simulink model "ConSys_A1"  (Simulink 8.3)
settings: Solver=ode3  StartTime=0.0  StopTime=Time(end)  FixedStep=Ts  RelTol=1e-3
values from neighbouring files (symbols this model uses):
  d = r*h    (= 1.6)    [StartUp_A1.m]
  d0 = d*h    (= 0.0032)    [StartUp_A1.m]
  h = 0.002    [StartUp_A1.m]
  Ka = diag([ 3  20  20  150  355  520])    [StartUp_A1.m]
  Kd = diag([ 3   5  25  100   15 1050])    [StartUp_A1.m]
  Ki = diag([35 555 810 7410 1850 5815])    [StartUp_A1.m]
  Kp = diag([55 180 350 1960  680 4450])    [StartUp_A1.m]
  r = 800    [StartUp_A1.m]
  TD = ss(Atd,Btd,Ctd,Dtd,Ts)    [StartUp_A1.m]
  Ts = 1/200    (= 0.005)    [StartUp_A1.m]
undefined symbols (not defined in the file or in its folder): DiscIntNeverNeededParam
undefined symbols (not defined in the file): ADAMS_cwd, ADAMS_exec, ADAMS_host, ADAMS_init, ADAMS_inputs, ADAMS_outputs, ADAMS_prefix, ADAMS_static, ADAMS_sysdir
libraries: cstblocks x6
(part 4 of 9)

== matlab function A2/MATLAB Function 1 ==
  data: q input double; V1 output double; dq input double
function V1 = V1(q,dq)
%#codegen
Th1=q(1,1); Th2=q(2,1); Th3=q(3,1); Th4=q(4,1); Th5=q(5,1); Th6=q(6,1);
dTh1=dq(1); dTh2=dq(2); dTh3=dq(3); dTh4=dq(4); dTh5=dq(5); dTh6=dq(6);
%---------------------------
V111=(0)*dTh1*dTh1;
V112=(0.09072*cos(2.0*Th2) + 1.0168*sin(2.0*Th2) + 0.01253*cos(2.0*Th2 + 2.0*Th3) - 0.69402*cos(Th2) - 2.7438*sin(2.0*Th2 + 2.0*Th3) + 0.034055*sin(Th2) + 0.19294*cos(Th2)^2 - 1.0*(1.108*sin(Th2 + Th3) + 4.68*cos(Th2) + 3.302*cos(Th2)*sin(Th3) + 3.302*cos(Th3)*sin(Th2))*(0.08523*cos(Th2 + Th3) - 0.36*sin(Th2) + 0.254*cos(Th2)*cos(Th3) - 0.254*sin(Th2)*sin(Th3) + 0.07) + (cos(Th6)*(sin(Th2 + Th3)*sin(Th5) - 1.0*cos(Th2 + Th3)*cos(Th4)*cos(Th5)) + cos(Th2 + Th3)*sin(Th4)*sin(Th6))*(0.001043*cos(Th6)*(cos(Th2 + Th3)*sin(Th5) + sin(Th2 + Th3)*cos(Th4)*cos(Th5)) - 4.0e-6*cos(Th2 + Th3)*cos(Th5) + 4.0e-6*sin(Th2 + Th3)*cos(Th4)*sin(Th5) - 0.001043*sin(Th2 + Th3)*sin(Th4)*sin(Th6)) + 0.009886*cos(Th2 + Th3)*sin(Th2 + Th3) + (sin(Th6)*(cos(Th2 + Th3)*sin(Th5) + sin(Th2 + Th3)*cos(Th4)*cos(Th5)) + sin(Th2 + Th3)*cos(Th6)*sin(Th4))*(0.00104*sin(Th6)*(sin(Th2 + Th3)*sin(Th5) - 1.0*cos(Th2 + Th3)*cos(Th4)*cos(Th5)) - 0.00104*cos(Th2 + Th3)*cos(Th6)*sin(Th4)) + (sin(Th6)*(sin(Th2 + Th3)*sin(Th5) - 1.0*cos(Th2 + Th3)*cos(Th4)*cos(Th5)) - 1.0*cos(Th2 + Th3)*cos(Th6)*sin(Th4))*(0.00104*sin(Th6)*(cos(Th2 + Th3)*sin(Th5) + sin(Th2 + Th3)*cos(Th4)*cos(Th5)) + 0.00104*sin(Th2 + Th3)*cos(Th6)*sin(Th4)) - 1.0*(sin(Th2 + Th3)*cos(Th5) + cos(Th2 + Th3)*cos(Th4)*sin(Th5))*(4.0e-6*cos(Th6)*(cos(Th2 + Th3)*sin(Th5) + sin(Th2 + Th3)*cos(Th4)*cos(Th5)) - 0.000116*cos(Th2 + Th3)*cos(Th5) + 0.000116*sin(Th2 + Th3)*cos(Th4)*sin(Th5) - 4.0e-6*sin(Th2 + Th3)*sin(Th4)*sin(Th6)) - 1.0*(cos(Th2 + Th3)*cos(Th5) - 1.0*sin(Th2 + Th3)*cos(Th4)*sin(Th5))*(4.0e-6*cos(Th6)*(sin(Th2 + Th3)*sin(Th5) - 1.0*cos(Th2 + Th3)*cos(Th4)*cos(Th5)) - 0.000116*sin(Th2 + Th3)*cos(Th5) - 0.000116*cos(Th2 + Th3)*cos(Th4)*sin(Th5) + 4.0e-6*cos(Th2 + Th3)*sin(Th4)*sin(Th6)) + (0.252*sin(Th2 + Th3) + 0.72*cos(Th2) + 0.00124*cos(Th2 + Th3)*sin(Th4) - 0.00304*sin(Th2 + Th3)*cos(Th5) - 0.00004*sin(Th2 + Th3)*sin(Th5) + 0.508*cos(Th2)*sin(Th3) + 0.508*cos(Th3)*sin(Th2) + 0.00004*cos(Th2 + Th3)*cos(Th4)*cos(Th5) - 0.00304*cos(Th2 + Th3)*cos(Th4)*sin(Th5))*(0.36*sin(Th2) - 0.126*cos(Th2 + Th3) + 0.00152*cos(Th2 + Th3)*cos(Th5) + 0.00002*cos(Th2 + Th3)*sin(Th5) + 0.00062*sin(Th2 + Th3)*sin(Th4) - 0.254*cos(Th2)*cos(Th3) + 0.254*sin(Th2)*sin(Th3) + 0.00002*sin(Th2 + Th3)*cos(Th4)*cos(Th5) - 0.00152*sin(Th2 + Th3)*cos(Th4)*sin(Th5) - 0.07) - 1.0*(0.126*sin(Th2 + Th3) + 0.36*cos(Th2) + 0.05206*sin(Th2 + Th3)*cos(Th5) + 0.254*cos(Th2)*sin(Th3) + 0.254*cos(Th3)*sin(Th2) + 0.05206*cos(Th2 + Th3)*cos(Th4)*sin(Th5) + 0.00023*cos(Th2 + Th3)*sin(Th4)*sin(Th6) + 0.00023*sin(Th2 + Th3)*cos(Th6)*sin(Th5) - 0.00023*cos(Th2 + Th3)*cos(Th4)*cos(Th5)*cos(Th6))*(0.126*cos(Th2 + Th3) - 0.36*sin(Th2) + 0.05206*cos(Th2 + Th3)*cos(Th5) + 0.254*cos(Th2)*cos(Th3) - 0.254*sin(Th2)*sin(Th3) + 0.00023*cos(Th2 + Th3)*cos(Th6)*sin(Th5) - 0.05206*sin(Th2 + Th3)*cos(Th4)*sin(Th5) - 0.00023*sin(Th2 + Th3)*sin(Th4)*sin(Th6) + 0.00023*sin(Th2 + Th3)*cos(Th4)*cos(Th5)*cos(Th6) + 0.07) - 1.0*(0.03204*cos(Th2 + Th3) + 4.9136*sin(Th2 + Th3) - 12.96*cos(Th2))*(0.13649*cos(Th2 + Th3) - 0.00089*sin(Th2 + Th3) + 0.36*sin(Th2) - 0.07) + 1.9612*cos(Th2)*sin(Th2) + (cos(Th6)*(cos(Th2 + Th3)*sin(Th5) + sin(Th2 + Th3)*cos(Th4)*cos(Th5)) - 1.0*sin(Th2 + Th3)*sin(Th4)*sin(Th6))*(0.001043*cos(Th6)*(sin(Th2 + Th3)*sin(Th5) - 1.0*cos(Th2 + Th3)*cos(Th4)*cos(Th5)) - 4.0e-6*sin(Th2 + Th3)*cos(Th5) - 4.0e-6*cos(Th2 + Th3)*cos(Th4)*sin(Th5) + 0.001043*cos(Th2 + Th3)*sin(Th4)*sin(Th6)) - 0.02225*cos(Th2 + Th3)*sin(Th2 + Th3)*cos(Th4)^2 + 0.000978*cos(Th2 + Th3)*sin(Th2 + Th3)*cos(Th5)^2 - 0.04182*cos(Th2 + Th3)*sin(Th2 + Th3)*sin(Th4)^2 + 0.009796*cos(Th2 + Th3)*sin(Th2 + Th3)*sin(Th5)^2 - 0.00008*cos(Th2 + Th3)^2*cos(Th5)*sin(Th4) + 0.00008*sin(Th2 + Th3)^2*cos(Th5)*sin(Th4) - 0.008818*cos(Th2 + Th3)^2*cos(Th4)*cos(Th5)*sin(Th5) + 0.008818*sin(Th2 + Th3)^2*cos(Th4)*cos(Th5)*sin(Th5) - 0.009796*cos(Th2 + Th3)*sin(Th2 + Th3)*cos(Th4)^2*cos(Th5)^2 - 0.000978*cos(Th2 + Th3)*sin(Th2 + Th3)*cos(Th4)^2*sin(Th5)^2 + 0.00016*cos(Th2 + Th3)*sin(Th2 + Th3)*cos(Th4)*sin(Th4)*sin(Th5) - 0.096468)*dTh1*dTh2;
V113=(0.01253*cos(2.0*Th2 + 2.0*Th3) - 2.7438*sin(2.0*Th2 + 2.0*Th3) - 1.0*(0.03204*cos(Th2 + Th3) + 4.9136*sin(Th2 + Th3))*(0.13649*cos(Th2 + Th3) - 0.00089*sin(Th2 + Th3) + 0.36*sin(Th2) - 0.07) + (cos(Th6)*(sin(Th2 + Th3)*sin(Th5) - 1.0*cos(Th2 + Th3)*cos(Th4)*cos(Th5)) + cos(Th2 + Th3)*sin(Th4)*sin(Th6))*(0.001043*cos(Th6)*(cos(Th2 + Th3)*sin(Th5) + sin(Th2 + Th3)*cos(Th4)*cos(Th5)) - 4.0e-6*cos(Th2 + Th3)*cos(Th5) + 4.0e-6*sin(Th2 + Th3)*cos(Th4)*sin(Th5) - 0.001043*sin(Th2 + Th3)*sin(Th4)*sin(Th6)) + (0.252*sin(Th2 + Th3) + 0.00124*cos(Th2 + Th3)*sin(Th4) - 0.00304*sin(Th2 + Th3)*cos(Th5) - 0.00004*sin(Th2 + Th3)*sin(Th5) + 0.508*cos(Th2)*sin(Th3) + 0.508*cos(Th3)*sin(Th2) + 0.00004*cos(Th2 + Th3)*cos(Th4)*cos(Th5) - 0.00304*cos(Th2 + Th3)*cos(Th4)*sin(Th5))*(0.36*sin(Th2) - 0.126*cos(Th2 + Th3) + 0.00152*cos(Th2 + Th3)*cos(Th5) + 0.00002*cos(Th2 + Th3)*sin(Th5) + 0.00062*sin(Th2 + Th3)*sin(Th4) - 0.254*cos(Th2)*cos(Th3) + 0.254*sin(Th2)*sin(Th3) + 0.00002*sin(Th2 + Th3)*cos(Th4)*cos(Th5) - 0.00152*sin(Th2 + Th3)*cos(Th4)*sin(Th5) - 0.07) - 1.0*(0.126*sin(Th2 + Th3) + 0.05206*sin(Th2 + Th3)*cos(Th5) + 0.254*cos(Th2)*sin(Th3) + 0.254*cos(Th3)*sin(Th2) + 0.05206*cos(Th2 + Th3)*cos(Th4)*sin(Th5) + 0.00023*cos(Th2 + Th3)*sin(Th4)*sin(Th6) + 0.00023*sin(Th2 + Th3)*cos(Th6)*sin(Th5) - 0.00023*cos(Th2 + Th3)*cos(Th4)*cos(Th5)*cos(Th6))*(0.126*cos(Th2 + Th3) - 0.36*sin(Th2) + 0.05206*cos(Th2 + Th3)*cos(Th5) + 0.254*cos(Th2)*cos(Th3) - 0.254*sin(Th2)*sin(Th3) + 0.00023*cos(Th2 + Th3)*cos(Th6)*sin(Th5) - 0.05206*sin(Th2 + Th3)*cos(Th4)*sin(Th5) - 0.00023*sin(Th2 + Th3)*sin(Th4)*sin(Th6) + 0.00023*sin(Th2 + Th3)*cos(Th4)*cos(Th5)*cos(Th6) + 0.07) + 0.009886*cos(Th2 + Th3)*sin(Th2 + Th3) + (sin(Th6)*(cos(Th2 + Th3)*sin(Th5) + sin(Th2 + Th3)*cos(Th4)*cos(Th5)) + sin(Th2 + Th3)*cos(Th6)*sin(Th4))*(0.00104*sin(Th6)*(sin(Th2 + Th3)*sin(Th5) - 1.0*cos(Th2 + Th3)*cos(Th4)*cos(Th5)) - 0.00104*cos(Th2 + Th3)*cos(Th6)*sin(Th4)) + (sin(Th6)*(sin(Th2 + Th3)*sin(Th5) - 1.0*cos(Th2 + Th3)*cos(Th4)*cos(Th5)) - 1.0*cos(Th2 + Th3)*cos(Th6)*sin(Th4))*(0.00104*sin(Th6)*(cos(Th2 + Th3)*sin(Th5) + sin(Th2 + Th3)*cos(Th4)*cos(Th5)) + 0.00104*sin(Th2 + Th3)*cos(Th6)*sin(Th4)) - 1.0*(sin(Th2 + Th3)*cos(Th5) + cos(Th2 + Th3)*cos(Th4)*sin(Th5))*(4.0e-6*cos(Th6)*(cos(Th2 + Th3)*sin(Th5) + sin(Th2 + Th3)*cos(Th4)*cos(Th5)) - 0.000116*cos(Th2 + Th3)*cos(Th5) + 0.000116*sin(Th2 + Th3)*cos(Th4)*sin(Th5) - 4.0e-6*sin(Th2 + Th3)*sin(Th4)*sin(Th6)) - 1.0*(cos(Th2 + Th3)*cos(Th5) - 1.0*sin(Th2 + Th3)*cos(Th4)*sin(Th5))*(4.0e-6*cos(Th6)*(sin(Th2 + Th3)*sin(Th5) - 1.0*cos(Th2 + Th3)*cos(Th4)*cos(Th5)) - 0.000116*sin(Th2 + Th3)*cos(Th5) - 0.000116*cos(Th2 + Th3)*cos(Th4)*sin(Th5) + 4.0e-6*cos(Th2 + Th3)*sin(Th4)*sin(Th6)) - 1.0*(1.108*sin(Th2 + Th3) + 3.302*cos(Th2)*sin(Th3) + 3.302*cos(Th3)*sin(Th2))*(0.08523*cos(Th2 + Th3) - 0.36*sin(Th2) + 0.254*cos(Th2)*cos(Th3) - 0.254*sin(Th2)*sin(Th3) + 0.07) + (cos(Th6)*(cos(Th2 + Th3)*sin(Th5) + sin(Th2 + Th3)*cos(Th4)*cos(Th5)) - 1.0*sin(Th2 + Th3)*sin(Th4)*sin(Th6))*(0.001043*cos(Th6)*(sin(Th2 + Th3)*sin(Th5) - 1.0*cos(Th2 + Th3)*cos(Th4)*cos(Th5)) - 4.0e-6*sin(Th2 + Th3)*cos(Th5) - 4.0e-6*cos(Th2 + Th3)*cos(Th4)*sin(Th5) + 0.001043*cos(Th2 + Th3)*sin(Th4)*sin(Th6)) - 0.02225*cos(Th2 + Th3)*sin(Th2 + Th3)*cos(Th4)^2 + 0.000978*cos(Th2 + Th3)*sin(Th2 + Th3)*cos(Th5)^2 - 0.04182*cos(Th2 + Th3)*sin(Th2 + Th3)*sin(Th4)^2 + 0.009796*cos(Th2 + Th3)*sin(Th2 + Th3)*sin(Th5)^2 - 0.00008*cos(Th2 + Th3)^2*cos(Th5)*sin(Th4) + 0.00008*sin(Th2 + Th3)^2*cos(Th5)*sin(Th4) - 0.008818*cos(Th2 + Th3)^2*cos(Th4)*cos(Th5)*sin(Th5) + 0.008818*sin(Th2 + Th3)^2*cos(Th4)*cos(Th5)*sin(Th5) - 0.009796*cos(Th2 + Th3)*sin(Th2 + Th3)*cos(Th4)^2*cos(Th5)^2 - 0.000978*cos(Th2 + Th3)*sin(Th2 + Th3)*cos(Th4)^2*sin(Th5)^2 + 0.00016*cos(Th2 + Th3)*sin(Th2 + Th3)*cos(Th4)*sin(Th4)*sin(Th5))*dTh1*dTh3;
V114=((0.00124*cos(Th4) - 0.00004*cos(Th5)*sin(Th4) + 0.00304*sin(Th4)*sin(Th5))*(0.00062*sin(Th2 + Th3)^2*sin(Th4) - 0.063*sin(2.0*Th2 + 2.0*Th3) - 0.00062*sin(Th4) - 0.07*sin(Th2 + Th3) + 0.36*sin(Th2 + Th3)*sin(Th2) - 0.00002*cos(Th4)*cos(Th5) + 0.00152*cos(Th4)*sin(Th5) + 0.00002*cos(Th2 + Th3)*sin(Th2 + Th3)*sin(Th5) - 0.254*sin(Th2 + Th3)*cos(Th2)*cos(Th3) + 0.254*sin(Th2 + Th3)*sin(Th2)*sin(Th3) + 0.00002*sin(Th2 + Th3)^2*cos(Th4)*cos(Th5) - 0.00152*sin(Th2 + Th3)^2*cos(Th4)*sin(Th5) + 0.00152*cos(Th2 + Th3)*sin(Th2 + Th3)*cos(Th5)) - 1.0*(0.00023*cos(Th4)*sin(Th6) - 0.05206*sin(Th4)*sin(Th5) + 0.00023*cos(Th5)*cos(Th6)*sin(Th4))*(0.07*sin(Th2 + Th3) + 0.063*sin(2.0*Th2 + 2.0*Th3) - 0.36*sin(Th2 + Th3)*sin(Th2) + 0.05206*cos(Th4)*sin(Th5) + 0.00023*sin(Th4)*sin(Th6) + 0.254*sin(Th2 + Th3)*cos(Th2)*cos(Th3) - 0.254*sin(Th2 + Th3)*sin(Th2)*sin(Th3) - 0.00023*cos(Th4)*cos(Th5)*cos(Th6) - 0.05206*sin(Th2 + Th3)^2*cos(Th4)*sin(Th5) - 0.00023*sin(Th2 + Th3)^2*sin(Th4)*sin(Th6) + 0.05206*cos(Th2 + Th3)*sin(Th2 + Th3)*cos(Th5) + 0.00023*sin(Th2 + Th3)^2*cos(Th4)*cos(Th5)*cos(Th6) + 0.00023*cos(Th2 + Th3)*sin(Th2 + Th3)*cos(Th6)*sin(Th5)) + 2.2737e-18*cos(Th2 + Th3)*(3.5184e13*cos(Th2 + Th3)*sin(Th5) + 4.1368e15*cos(Th2 + Th3)*cos(Th4)*sin(Th4) - 3.5184e13*sin(Th2 + Th3)*cos(Th4)*cos(Th5) - 7.0369e13*cos(Th2 + Th3)*cos(Th4)^2*sin(Th5) + 3.8782e15*sin(Th2 + Th3)*cos(Th5)*sin(Th4)*sin(Th5) - 3.8782e15*cos(Th2 + Th3)*cos(Th4)*cos(Th5)^2*sin(Th4)) + 8.4703e-22*cos(Th2 + Th3)*(1.2314e18*cos(Th4)*sin(Th6) + 4.7224e15*sin(Th4)*sin(Th5) + 1.2314e18*cos(Th5)*cos(Th6)*sin(Th4))*(cos(Th2 + Th3)*sin(Th4)*sin(Th6) + sin(Th2 + Th3)*cos(Th6)*sin(Th5) - 1.0*cos(Th2 + Th3)*cos(Th4)*cos(Th5)*cos(Th6)) + 0.00104*cos(Th2 + Th3)*(cos(Th4)*cos(Th6) - 1.0*cos(Th5)*sin(Th4)*sin(Th6))*(cos(Th2 + Th3)*cos(Th6)*sin(Th4) - 1.0*sin(Th2 + Th3)*sin(Th5)*sin(Th6) + cos(Th2 + Th3)*cos(Th4)*cos(Th5)*sin(Th6)) + 0.009186*cos(Th2 + Th3)^2*cos(Th4)*sin(Th4) + cos(Th2 + Th3)*(cos(Th4)*cos(Th6) - 1.0*cos(Th5)*sin(Th4)*sin(Th6))*(0.00104*cos(Th2 + Th3)*cos(Th6)*sin(Th4) - 0.00104*sin(Th2 + Th3)*sin(Th5)*sin(Th6) + 0.00104*cos(Th2 + Th3)*cos(Th4)*cos(Th5)*sin(Th6)) - 1.0*cos(Th2 + Th3)*(cos(Th4)*sin(Th6) + cos(Th5)*cos(Th6)*sin(Th4))*(4.0e-6*sin(Th2 + Th3)*cos(Th5) + 4.0e-6*cos(Th2 + Th3)*cos(Th4)*sin(Th5) - 0.001043*cos(Th2 + Th3)*sin(Th4)*sin(Th6) - 0.001043*sin(Th2 + Th3)*cos(Th6)*sin(Th5) + 0.001043*cos(Th2 + Th3)*cos(Th4)*cos(Th5)*cos(Th6)) - 8.4703e-22*cos(Th2 + Th3)*(sin(Th2 + Th3)*cos(Th5) + cos(Th2 + Th3)*cos(Th4)*sin(Th5))*(4.7224e15*cos(Th4)*sin(Th6) + 1.3695e17*sin(Th4)*sin(Th5) + 4.7224e15*cos(Th5)*cos(Th6)*sin(Th4)) - 1.0*cos(Th2 + Th3)*sin(Th4)*sin(Th5)*(0.000116*sin(Th2 + Th3)*cos(Th5) + 0.000116*cos(Th2 + Th3)*cos(Th4)*sin(Th5) - 4.0e-6*cos(Th2 + Th3)*sin(Th4)*sin(Th6) - 4.0e-6*sin(Th2 + Th3)*cos(Th6)*sin(Th5) + 4.0e-6*cos(Th2 + Th3)*cos(Th4)*cos(Th5)*cos(Th6)))*dTh1*dTh4;
V115=((cos(Th6)*(sin(Th2 + Th3)*sin(Th5) - 1.0*cos(Th2 + Th3)*cos(Th4)*cos(Th5)) + cos(Th2 + Th3)*sin(Th4)*sin(Th6))*(0.001043*cos(Th6)*(sin(Th2 + Th3)*cos(Th5) + cos(Th2 + Th3)*cos(Th4)*sin(Th5)) + 4.0e-6*sin(Th2 + Th3)*sin(Th5) - 4.0e-6*cos(Th2 + Th3)*cos(Th4)*cos(Th5)) - 1.0*(sin(Th2 + Th3)*cos(Th5) + cos(Th2 + Th3)*cos(Th4)*sin(Th5))*(4.0e-6*cos(Th6)*(sin(Th2 + Th3)*cos(Th5) + cos(Th2 + Th3)*cos(Th4)*sin(Th5)) + 0.000116*sin(Th2 + Th3)*sin(Th5) - 0.000116*cos(Th2 + Th3)*cos(Th4)*cos(Th5)) + (sin(Th2 + Th3)*sin(Th5) - 1.0*cos(Th2 + Th3)*cos(Th4)*cos(Th5))*(4.0e-6*cos(Th6)*(sin(Th2 + Th3)*sin(Th5) - 1.0*cos(Th2 + Th3)*cos(Th4)*cos(Th5)) - 0.000116*sin(Th2 + Th3)*cos(Th5) - 0.000116*cos(Th2 + Th3)*cos(Th4)*sin(Th5) + 4.0e-6*cos(Th2 + Th3)*sin(Th4)*sin(Th6)) + (0.00023*cos(Th6)*(sin(Th5)*(sin(Th1)*sin(Th4) - 1.0*sin(Th2 + Th3)*cos(Th1)*cos(Th4)) + cos(Th2 + Th3)*cos(Th1)*cos(Th5)) + 0.05206*cos(Th5)*(sin(Th1)*sin(Th4) - 1.0*sin(Th2 + Th3)*cos(Th1)*cos(Th4)) - 0.05206*cos(Th2 + Th3)*cos(Th1)*sin(Th5))*(0.07*cos(Th1) + 0.05206*sin(Th5)*(sin(Th1)*sin(Th4) - 1.0*sin(Th2 + Th3)*cos(Th1)*cos(Th4)) + 0.126*cos(Th2 + Th3)*cos(Th1) - 0.00023*sin(Th6)*(cos(Th4)*sin(Th1) + sin(Th2 + Th3)*cos(Th1)*sin(Th4)) - 0.36*cos(Th1)*sin(Th2) - 0.00023*cos(Th6)*(cos(Th5)*(sin(Th1)*sin(Th4) - 1.0*sin(Th2 + Th3)*cos(Th1)*cos(Th4)) - 1.0*cos(Th2 + Th3)*cos(Th1)*sin(Th5)) + 0.05206*cos(Th2 + Th3)*cos(Th1)*cos(Th5) + 0.254*cos(Th1)*cos(Th2)*cos(Th3) - 0.254*cos(Th1)*sin(Th2)*sin(Th3)) - 1.0*(0.00304*cos(Th5)*(cos(Th1)*sin(Th4) + sin(Th2 + Th3)*cos(Th4)*sin(Th1)) + 0.00004*sin(Th5)*(cos(Th1)*sin(Th4) + sin(Th2 + Th3)*cos(Th4)*sin(Th1)) - 0.00004*cos(Th2 + Th3)*cos(Th5)*sin(Th1) + 0.00304*cos(Th2 + Th3)*sin(Th1)*sin(Th5))*(0.00002*cos(Th5)*(cos(Th1)*sin(Th4) + sin(Th2 + Th3)*cos(Th4)*sin(Th1)) - 0.126*cos(Th2 + Th3)*sin(Th1) - 0.07*sin(Th1) - 0.00152*sin(Th5)*(cos(Th1)*sin(Th4) + sin(Th2 + Th3)*cos(Th4)*sin(Th1)) - 0.00062*cos(Th1)*cos(Th4) + 0.36*sin(Th1)*sin(Th2) + 0.00152*cos(Th2 + Th3)*cos(Th5)*sin(Th1) + 0.00002*cos(Th2 + Th3)*sin(Th1)*sin(Th5) + 0.00062*sin(Th2 + Th3)*sin(Th1)*sin(Th4) - 0.254*cos(Th2)*cos(Th3)*sin(Th1) + 0.254*sin(Th1)*sin(Th2)*sin(Th3)) + (0.00304*cos(Th5)*(sin(Th1)*sin(Th4) - 1.0*sin(Th2 + Th3)*cos(Th1)*cos(Th4)) + 0.00004*sin(Th5)*(sin(Th1)*sin(Th4) - 1.0*sin(Th2 + Th3)*cos(Th1)*cos(Th4)) + 0.00004*cos(Th2 + Th3)*cos(Th1)*cos(Th5) - 0.00304*cos(Th2 + Th3)*cos(Th1)*sin(Th5))*(0.00152*sin(Th5)*(sin(Th1)*sin(Th4) - 1.0*sin(Th2 + Th3)*cos(Th1)*cos(Th4)) - 0.00002*cos(Th5)*(sin(Th1)*sin(Th4) - 1.0*sin(Th2 + Th3)*cos(Th1)*cos(Th4)) - 0.07*cos(Th1) - 0.126*cos(Th2 + Th3)*cos(Th1) + 0.36*cos(Th1)*sin(Th2) + 0.00062*cos(Th4)*sin(Th1) + 0.00152*cos(Th2 + Th3)*cos(Th1)*cos(Th5) + 0.00002*cos(Th2 + Th3)*cos(Th1)*sin(Th5) + 0.00062*sin(Th2 + Th3)*cos(Th1)*sin(Th4) - 0.254*cos(Th1)*cos(Th2)*cos(Th3) + 0.254*cos(Th1)*sin(Th2)*sin(Th3)) - 1.0*(0.00023*cos(Th6)*(sin(Th5)*(cos(Th1)*sin(Th4) + sin(Th2 + Th3)*cos(Th4)*sin(Th1)) - 1.0*cos(Th2 + Th3)*cos(Th5)*sin(Th1)) + 0.05206*cos(Th5)*(cos(Th1)*sin(Th4) + sin(Th2 + Th3)*cos(Th4)*sin(Th1)) + 0.05206*cos(Th2 + Th3)*sin(Th1)*sin(Th5))*(0.07*sin(Th1) + 0.00023*sin(Th6)*(cos(Th1)*cos(Th4) - 1.0*sin(Th2 + Th3)*sin(Th1)*sin(Th4)) + 0.00023*cos(Th6)*(cos(Th5)*(cos(Th1)*sin(Th4) + sin(Th2 + Th3)*cos(Th4)*sin(Th1)) + cos(Th2 + Th3)*sin(Th1)*sin(Th5)) + 0.126*cos(Th2 + Th3)*sin(Th1) - 0.05206*sin(Th5)*(cos(Th1)*sin(Th4) + sin(Th2 + Th3)*cos(Th4)*sin(Th1)) - 0.36*sin(Th1)*sin(Th2) + 0.05206*cos(Th2 + Th3)*cos(Th5)*sin(Th1) + 0.254*cos(Th2)*cos(Th3)*sin(Th1) - 0.254*sin(Th1)*sin(Th2)*sin(Th3)) + cos(Th6)*(sin(Th2 + Th3)*cos(Th5) + cos(Th2 + Th3)*cos(Th4)*sin(Th5))*(0.001043*cos(Th6)*(sin(Th2 + Th3)*sin(Th5) - 1.0*cos(Th2 + Th3)*cos(Th4)*cos(Th5)) - 4.0e-6*sin(Th2 + Th3)*cos(Th5) - 4.0e-6*cos(Th2 + Th3)*cos(Th4)*sin(Th5) + 0.001043*cos(Th2 + Th3)*sin(Th4)*sin(Th6)) + sin(Th6)*(sin(Th2 + Th3)*cos(Th5) + cos(Th2 + Th3)*cos(Th4)*sin(Th5))*(0.00104*sin(Th6)*(sin(Th2 + Th3)*sin(Th5) - 1.0*cos(Th2 + Th3)*cos(Th4)*cos(Th5)) - 0.00104*cos(Th2 + Th3)*cos(Th6)*sin(Th4)) + 0.008818*sin(Th2 + Th3)^2*cos(Th5)*sin(Th5) + 0.00104*sin(Th6)*(sin(Th2 + Th3)*cos(Th5) + cos(Th2 + Th3)*cos(Th4)*sin(Th5))*(sin(Th6)*(sin(Th2 + Th3)*sin(Th5) - 1.0*cos(Th2 + Th3)*cos(Th4)*cos(Th5)) - 1.0*cos(Th2 + Th3)*cos(Th6)*sin(Th4)) - 0.008818*cos(Th2 + Th3)*sin(Th2 + Th3)*cos(Th4)*cos(Th5)^2 + 0.008818*cos(Th2 + Th3)*sin(Th2 + Th3)*cos(Th4)*sin(Th5)^2 - 0.00008*cos(Th2 + Th3)^2*cos(Th4)*cos(Th5)*sin(Th4) - 0.008818*cos(Th2 + Th3)^2*cos(Th4)^2*cos(Th5)*sin(Th5) + 0.00008*cos(Th2 + Th3)*sin(Th2 + Th3)*sin(Th4)*sin(Th5))*dTh1*dTh5;
V116=(1.0*(0.00023*cos(Th6)*(cos(Th1)*cos(Th4) - 1.0*sin(Th2 + Th3)*sin(Th1)*sin(Th4)) - 0.00023*sin(Th6)*(cos(Th5)*(cos(Th1)*sin(Th4) + sin(Th2 + Th3)*cos(Th4)*sin(Th1)) + cos(Th2 + Th3)*sin(Th1)*sin(Th5)))*(0.07*sin(Th1) + 0.00023*sin(Th6)*(cos(Th1)*cos(Th4) - 1.0*sin(Th2 + Th3)*sin(Th1)*sin(Th4)) + 0.00023*cos(Th6)*(cos(Th5)*(cos(Th1)*sin(Th4) + sin(Th2 + Th3)*cos(Th4)*sin(Th1)) + cos(Th2 + Th3)*sin(Th1)*sin(Th5)) + 0.126*cos(Th2 + Th3)*sin(Th1) - 0.05206*sin(Th5)*(cos(Th1)*sin(Th4) + sin(Th2 + Th3)*cos(Th4)*sin(Th1)) - 0.36*sin(Th1)*sin(Th2) + 0.05206*cos(Th2 + Th3)*cos(Th5)*sin(Th1) + 0.254*cos(Th2)*cos(Th3)*sin(Th1) - 0.254*sin(Th1)*sin(Th2)*sin(Th3)) + (0.00104*cos(Th6)*(sin(Th2 + Th3)*sin(Th5) - 1.0*cos(Th2 + Th3)*cos(Th4)*cos(Th5)) + 0.00104*cos(Th2 + Th3)*sin(Th4)*sin(Th6))*(sin(Th6)*(sin(Th2 + Th3)*sin(Th5) - 1.0*cos(Th2 + Th3)*cos(Th4)*cos(Th5)) - 1.0*cos(Th2 + Th3)*cos(Th6)*sin(Th4)) + (sin(Th2 + Th3)*cos(Th5) + cos(Th2 + Th3)*cos(Th4)*sin(Th5))*(4.0e-6*sin(Th6)*(sin(Th2 + Th3)*sin(Th5) - 1.0*cos(Th2 + Th3)*cos(Th4)*cos(Th5)) - 4.0e-6*cos(Th2 + Th3)*cos(Th6)*sin(Th4)) - 1.0*(sin(Th6)*(sin(Th2 + Th3)*sin(Th5) - 1.0*cos(Th2 + Th3)*cos(Th4)*cos(Th5)) - 1.0*cos(Th2 + Th3)*cos(Th6)*sin(Th4))*(0.001043*cos(Th6)*(sin(Th2 + Th3)*sin(Th5) - 1.0*cos(Th2 + Th3)*cos(Th4)*cos(Th5)) - 4.0e-6*sin(Th2 + Th3)*cos(Th5) - 4.0e-6*cos(Th2 + Th3)*cos(Th4)*sin(Th5) + 0.001043*cos(Th2 + Th3)*sin(Th4)*sin(Th6)) + (0.00023*sin(Th6)*(cos(Th5)*(sin(Th1)*sin(Th4) - 1.0*sin(Th2 + Th3)*cos(Th1)*cos(Th4)) - 1.0*cos(Th2 + Th3)*cos(Th1)*sin(Th5)) - 0.00023*cos(Th6)*(cos(Th4)*sin(Th1) + sin(Th2 + Th3)*cos(Th1)*sin(Th4)))*(0.07*cos(Th1) + 0.05206*sin(Th5)*(sin(Th1)*sin(Th4) - 1.0*sin(Th2 + Th3)*cos(Th1)*cos(Th4)) + 0.126*cos(Th2 + Th3)*cos(Th1) - 0.00023*sin(Th6)*(cos(Th4)*sin(Th1) + sin(Th2 + Th3)*cos(Th1)*sin(Th4)) - 0.36*cos(Th1)*sin(Th2) - 0.00023*cos(Th6)*(cos(Th5)*(sin(Th1)*sin(Th4) - 1.0*sin(Th2 + Th3)*cos(Th1)*cos(Th4)) - 1.0*cos(Th2 + Th3)*cos(Th1)*sin(Th5)) + 0.05206*cos(Th2 + Th3)*cos(Th1)*cos(Th5) + 0.254*cos(Th1)*cos(Th2)*cos(Th3) - 0.254*cos(Th1)*sin(Th2)*sin(Th3)) + (0.00104*sin(Th6)*(sin(Th2 + Th3)*sin(Th5) - 1.0*cos(Th2 + Th3)*cos(Th4)*cos(Th5)) - 0.00104*cos(Th2 + Th3)*cos(Th6)*sin(Th4))*(cos(Th6)*(sin(Th2 + Th3)*sin(Th5) - 1.0*cos(Th2 + Th3)*cos(Th4)*cos(Th5)) + cos(Th2 + Th3)*sin(Th4)*sin(Th6)) - 1.0*(0.001043*sin(Th6)*(sin(Th2 + Th3)*sin(Th5) - 1.0*cos(Th2 + Th3)*cos(Th4)*cos(Th5)) - 0.001043*cos(Th2 + Th3)*cos(Th6)*sin(Th4))*(cos(Th6)*(sin(Th2 + Th3)*sin(Th5) - 1.0*cos(Th2 + Th3)*cos(Th4)*cos(Th5)) + cos(Th2 + Th3)*sin(Th4)*sin(Th6)))*dTh1*dTh6;
%---------------------------
V121=(0)*dTh2*dTh1;
V122=(0.039618*cos(Th2 + Th3) - 0.00015211*sin(Th2 + Th3) + 0.0017066*cos(Th2) + 0.71642*sin(Th2) - 1.0*(0.00062*cos(Th4) - 0.00002*cos(Th5)*sin(Th4) + 0.00152*sin(Th4)*sin(Th5))*(0.36*sin(Th2) - 0.126*cos(Th2 + Th3) + 0.00152*cos(Th2 + Th3)*cos(Th5) + 0.00002*cos(Th2 + Th3)*sin(Th5) + 0.00062*sin(Th2 + Th3)*sin(Th4) - 0.254*cos(Th2)*cos(Th3) + 0.254*sin(Th2)*sin(Th3) + 0.00002*sin(Th2 + Th3)*cos(Th4)*cos(Th5) - 0.00152*sin(Th2 + Th3)*cos(Th4)*sin(Th5)) + 0.00004*sin(Th2 + Th3)*sin(Th5) + (0.000115*cos(Th4)*sin(Th6) - 0.02603*sin(Th4)*sin(Th5) + 0.000115*cos(Th5)*cos(Th6)*sin(Th4))*(0.126*cos(Th2 + Th3) - 0.36*sin(Th2) + 0.05206*cos(Th2 + Th3)*cos(Th5) + 0.254*cos(Th2)*cos(Th3) - 0.254*sin(Th2)*sin(Th3) + 0.00023*cos(Th2 + Th3)*cos(Th6)*sin(Th5) - 0.05206*sin(Th2 + Th3)*cos(Th4)*sin(Th5) - 0.00023*sin(Th2 + Th3)*sin(Th4)*sin(Th6) + 0.00023*sin(Th2 + Th3)*cos(Th4)*cos(Th5)*cos(Th6)) + 0.00004*cos(Th2 + Th3)*cos(Th4)*cos(Th5) - 4.0e-6*cos(Th2 + Th3)*cos(Th6)*sin(Th4) + 0.010223*sin(Th2 + Th3)*cos(Th4)*sin(Th4) + 4.0e-6*sin(Th2 + Th3)*sin(Th5)*sin(Th6) - 0.00008*sin(Th2 + Th3)*cos(Th4)^2*sin(Th5) + 4.0e-6*cos(Th2 + Th3)*cos(Th4)*cos(Th5)*sin(Th6) - 0.005333*cos(Th2 + Th3)*cos(Th5)*sin(Th4)*sin(Th5) + 3.0e-6*sin(Th2 + Th3)*cos(Th5)*cos(Th6)*sin(Th6) + 8.0e-6*cos(Th2 + Th3)*cos(Th5)^2*cos(Th6)*sin(Th4) - 0.005333*sin(Th2 + Th3)*cos(Th4)*cos(Th5)^2*sin(Th4) - 3.0e-6*sin(Th2 + Th3)*cos(Th4)*cos(Th6)^2*sin(Th4) - 8.0e-6*sin(Th2 + Th3)*cos(Th4)^2*sin(Th5)*sin(Th6) - 3.0e-6*cos(Th2 + Th3)*cos(Th5)*cos(Th6)^2*sin(Th4)*sin(Th5) - 6.0e-6*sin(Th2 + Th3)*cos(Th4)^2*cos(Th5)*cos(Th6)*sin(Th6) - 3.0e-6*sin(Th2 + Th3)*cos(Th4)*cos(Th5)^2*cos(Th6)^2*sin(Th4) - 3.0e-6*cos(Th2 + Th3)*cos(Th4)*cos(Th6)*sin(Th5)*sin(Th6) - 8.0e-6*sin(Th2 + Th3)*cos(Th4)*cos(Th5)*cos(Th6)*sin(Th4)*sin(Th5))*dTh2*dTh2;
O123=0.039618*cos(Th2 + Th3) - 0.00015211*sin(Th2 + Th3) - 1.0*(0.00062*cos(Th4) - 0.00002*cos(Th5)*sin(Th4) + 0.00152*sin(Th4)*sin(Th5))*(0.00152*cos(Th2 + Th3)*cos(Th5) - 0.126*cos(Th2 + Th3) + 0.00002*cos(Th2 + Th3)*sin(Th5) + 0.00062*sin(Th2 + Th3)*sin(Th4) - 0.254*cos(Th2)*cos(Th3) + 0.254*sin(Th2)*sin(Th3) + 0.00002*sin(Th2 + Th3)*cos(Th4)*cos(Th5) - 0.00152*sin(Th2 + Th3)*cos(Th4)*sin(Th5)) + 0.00004*sin(Th2 + Th3)*sin(Th5) + (0.000115*cos(Th4)*sin(Th6) - 0.02603*sin(Th4)*sin(Th5) + 0.000115*cos(Th5)*cos(Th6)*sin(Th4))*(0.126*cos(Th2 + Th3) + 0.05206*cos(Th2 + Th3)*cos(Th5) + 0.254*cos(Th2)*cos(Th3) - 0.254*sin(Th2)*sin(Th3) + 0.00023*cos(Th2 + Th3)*cos(Th6)*sin(Th5) - 0.05206*sin(Th2 + Th3)*cos(Th4)*sin(Th5) - 0.00023*sin(Th2 + Th3)*sin(Th4)*sin(Th6) + 0.00023*sin(Th2 + Th3)*cos(Th4)*cos(Th5)*cos(Th6)) + 0.00004*cos(Th2 + Th3)*cos(Th4)*cos(Th5) - 4.0e-6*cos(Th2 + Th3)*cos(Th6)*sin(Th4) + 0.010223*sin(Th2 + Th3)*cos(Th4)*sin(Th4) + 4.0e-6*sin(Th2 + Th3)*sin(Th5)*sin(Th6) - 0.00008*sin(Th2 + Th3)*cos(Th4)^2*sin(Th5) + 4.0e-6*cos(Th2 + Th3)*cos(Th4)*cos(Th5)*sin(Th6) - 0.005333*cos(Th2 + Th3)*cos(Th5)*sin(Th4)*sin(Th5) + 3.0e-6*sin(Th2 + Th3)*cos(Th5)*cos(Th6)*sin(Th6) + 8.0e-6*cos(Th2 + Th3)*cos(Th5)^2*cos(Th6)*sin(Th4) - 0.005333*sin(Th2 + Th3)*cos(Th4)*cos(Th5)^2*sin(Th4) - 3.0e-6*sin(Th2 + Th3)*cos(Th4)*cos(Th6)^2*sin(Th4) - 8.0e-6*sin(Th2 + Th3)*cos(Th4)^2*sin(Th5)*sin(Th6) - 3.0e-6*cos(Th2 + Th3)*cos(Th5)*cos(Th6)^2*sin(Th4)*sin(Th5) - 6.0e-6*sin(Th2 + Th3)*cos(Th4)^2*cos(Th5)*cos(Th6)*sin(Th6) - 3.0e-6*sin(Th2 + Th3)*cos(Th4)*cos(Th5)^2*cos(Th6)^2*sin(Th4) - 3.0e-6*cos(Th2 + Th3)*cos(Th4)*cos(Th6)*sin(Th5)*sin(Th6) - 8.0e-6*sin(Th2 + Th3)*cos(Th4)*cos(Th5)*cos(Th6)*sin(Th4)*sin(Th5);
V123=O123*dTh2*dTh3;
V124=(0.010223*cos(Th2 + Th3) + 5.0e-11*cos(Th2 + Th3)*(23.0*cos(Th4)*sin(Th6) - 5206.0*sin(Th4)*sin(Th5) + 23.0*cos(Th5)*cos(Th6)*sin(Th4))^2 - 1.0*(0.02603*cos(Th4)*sin(Th5) + 0.000115*sin(Th4)*sin(Th6) - 0.000115*cos(Th4)*cos(Th5)*cos(Th6))*(0.126*sin(Th2 + Th3) + 0.36*cos(Th2) + 0.05206*sin(Th2 + Th3)*cos(Th5) + 0.254*cos(Th2)*sin(Th3) + 0.254*cos(Th3)*sin(Th2) + 0.05206*cos(Th2 + Th3)*cos(Th4)*sin(Th5) + 0.00023*cos(Th2 + Th3)*sin(Th4)*sin(Th6) + 0.00023*sin(Th2 + Th3)*cos(Th6)*sin(Th5) - 0.00023*cos(Th2 + Th3)*cos(Th4)*cos(Th5)*cos(Th6)) - 1.0*(0.00062*sin(Th4) + 0.00002*cos(Th4)*cos(Th5) - 0.00152*cos(Th4)*sin(Th5))*(0.126*sin(Th2 + Th3) + 0.36*cos(Th2) + 0.00062*cos(Th2 + Th3)*sin(Th4) - 0.00152*sin(Th2 + Th3)*cos(Th5) - 0.00002*sin(Th2 + Th3)*sin(Th5) + 0.254*cos(Th2)*sin(Th3) + 0.254*cos(Th3)*sin(Th2) + 0.00002*cos(Th2 + Th3)*cos(Th4)*cos(Th5) - 0.00152*cos(Th2 + Th3)*cos(Th4)*sin(Th5)) - 0.020446*cos(Th2 + Th3)*cos(Th4)^2 - 0.005333*cos(Th2 + Th3)*cos(Th5)^2 - 3.0e-6*cos(Th2 + Th3)*cos(Th6)^2 + 4.0e-10*cos(Th2 + Th3)*(31.0*cos(Th4) - 1.0*cos(Th5)*sin(Th4) + 76.0*sin(Th4)*sin(Th5))^2 - 4.0e-6*sin(Th2 + Th3)*cos(Th4)*cos(Th6) - 0.00004*sin(Th2 + Th3)*cos(Th5)*sin(Th4) + 0.010666*cos(Th2 + Th3)*cos(Th4)^2*cos(Th5)^2 + 6.0e-6*cos(Th2 + Th3)*cos(Th4)^2*cos(Th6)^2 - 3.0e-6*cos(Th2 + Th3)*cos(Th5)^2*cos(Th6)^2 - 8.0e-6*cos(Th2 + Th3)*cos(Th5)*cos(Th6)*sin(Th5) + 6.0e-6*cos(Th2 + Th3)*cos(Th4)^2*cos(Th5)^2*cos(Th6)^2 - 0.00016*cos(Th2 + Th3)*cos(Th4)*sin(Th4)*sin(Th5) - 0.005333*sin(Th2 + Th3)*cos(Th4)*cos(Th5)*sin(Th5) - 4.0e-6*sin(Th2 + Th3)*cos(Th5)*sin(Th4)*sin(Th6) + 8.0e-6*sin(Th2 + Th3)*cos(Th4)*cos(Th5)^2*cos(Th6) + 0.000016*cos(Th2 + Th3)*cos(Th4)^2*cos(Th5)*cos(Th6)*sin(Th5) - 3.0e-6*sin(Th2 + Th3)*cos(Th4)*cos(Th5)*cos(Th6)^2*sin(Th5) - 0.000016*cos(Th2 + Th3)*cos(Th4)*sin(Th4)*sin(Th5)*sin(Th6) + 3.0e-6*sin(Th2 + Th3)*cos(Th6)*sin(Th4)*sin(Th5)*sin(Th6) - 0.000012*cos(Th2 + Th3)*cos(Th4)*cos(Th5)*cos(Th6)*sin(Th4)*sin(Th6))*dTh2*dTh4;
V125=(0.005333*sin(Th2 + Th3)*sin(Th4) - 0.00004*cos(Th2 + Th3)*cos(Th5) - 1.24e-8*sin(Th2 + Th3)*cos(Th4)*cos(Th5) - 4.0e-6*cos(Th2 + Th3)*cos(Th5)*sin(Th6) - 0.000039058*sin(Th2 + Th3)*cos(Th4)*sin(Th5) - 0.0030883*sin(Th2 + Th3)*cos(Th5)*sin(Th4) + 2.52e-6*sin(Th2 + Th3)*sin(Th4)*sin(Th5) - 0.0088236*cos(Th2)*cos(Th5)*sin(Th4) + 0.000079058*cos(Th2 + Th3)*cos(Th4)^2*cos(Th5) + 7.2e-6*cos(Th2)*sin(Th4)*sin(Th5) + 9.424e-7*cos(Th2 + Th3)*cos(Th5)*sin(Th4)^2 - 1.24e-8*cos(Th2 + Th3)*cos(Th4)^2*sin(Th5) + 1.24e-8*cos(Th2 + Th3)*sin(Th4)^2*sin(Th5) - 0.012023*sin(Th2 + Th3)*cos(Th5)^2*sin(Th4) + 3.0e-6*sin(Th2 + Th3)*cos(Th6)^2*sin(Th4) + 0.0013574*sin(Th2 + Th3)*sin(Th4)*sin(Th5)^2 - 8.0e-6*cos(Th2 + Th3)*cos(Th4)*cos(Th6)*sin(Th4) + 3.0e-6*cos(Th2 + Th3)*cos(Th6)*sin(Th5)*sin(Th6) - 1.216e-7*sin(Th2 + Th3)*cos(Th5)*sin(Th4)*sin(Th5) - 9.9869e-6*sin(Th2 + Th3)*cos(Th4)*sin(Th5)*sin(Th6) - 0.00001449*sin(Th2 + Th3)*cos(Th6)*sin(Th4)*sin(Th5) - 0.0062255*cos(Th2)*cos(Th5)*sin(Th3)*sin(Th4) - 0.0062255*cos(Th3)*cos(Th5)*sin(Th2)*sin(Th4) - 0.0000414*cos(Th2)*cos(Th6)*sin(Th4)*sin(Th5) + 6.08e-8*cos(Th2 + Th3)*cos(Th4)*cos(Th5)^2*sin(Th4) + 0.000013987*cos(Th2 + Th3)*cos(Th4)^2*cos(Th5)*sin(Th6) + 5.08e-6*cos(Th2)*sin(Th3)*sin(Th4)*sin(Th5) + 5.08e-6*cos(Th3)*sin(Th2)*sin(Th4)*sin(Th5) - 6.08e-8*cos(Th2 + Th3)*cos(Th4)*sin(Th4)*sin(Th5)^2 - 5.9869e-6*cos(Th2 + Th3)*cos(Th5)*sin(Th4)^2*sin(Th6) - 5.9735e-6*sin(Th2 + Th3)*cos(Th5)^2*cos(Th6)^2*sin(Th4) - 2.645e-8*sin(Th2 + Th3)*cos(Th6)^2*sin(Th4)*sin(Th5)^2 + 0.000027974*cos(Th2 + Th3)*cos(Th4)*cos(Th5)^2*cos(Th6)*sin(Th4) - 0.00002921*cos(Th2)*cos(Th6)*sin(Th3)*sin(Th4)*sin(Th5) - 0.00002921*cos(Th3)*cos(Th6)*sin(Th2)*sin(Th4)*sin(Th5) - 0.000011974*cos(Th2 + Th3)*cos(Th4)*cos(Th6)*sin(Th4)*sin(Th5)^2 - 5.9735e-6*cos(Th2 + Th3)*cos(Th4)^2*cos(Th6)*sin(Th5)*sin(Th6) - 2.645e-8*cos(Th2 + Th3)*cos(Th6)*sin(Th4)^2*sin(Th5)*sin(Th6) - 0.013381*cos(Th2 + Th3)*cos(Th4)*cos(Th5)*sin(Th4)*sin(Th5) - 2.9736e-6*sin(Th2 + Th3)*cos(Th4)*cos(Th5)*cos(Th6)*sin(Th6) - 0.000039948*sin(Th2 + Th3)*cos(Th5)*cos(Th6)*sin(Th4)*sin(Th5) - 5.9471e-6*cos(Th2 + Th3)*cos(Th4)*cos(Th5)*cos(Th6)^2*sin(Th4)*sin(Th5))*dTh2*dTh5;
V126=(3.0e-6*cos(Th2 + Th3)*cos(Th5) + 0.00001449*sin(Th2 + Th3)*cos(Th4)*cos(Th6) - 4.0e-6*cos(Th2 + Th3)*cos(Th6)*sin(Th5) + 3.0e-6*sin(Th2 + Th3)*cos(Th4)*sin(Th5) + 4.0e-6*sin(Th2 + Th3)*sin(Th4)*sin(Th6) + 0.0000414*cos(Th2)*cos(Th4)*cos(Th6) - 6.0e-6*cos(Th2 + Th3)*cos(Th4)^2*cos(Th5) - 6.0e-6*cos(Th2 + Th3)*cos(Th5)*cos(Th6)^2 + 9.9869e-6*sin(Th2 + Th3)*cos(Th4)*cos(Th5)*cos(Th6) - 0.00001449*sin(Th2 + Th3)*cos(Th5)*sin(Th4)*sin(Th6) + 0.00002921*cos(Th2)*cos(Th4)*cos(Th6)*sin(Th3) + 0.00002921*cos(Th3)*cos(Th4)*cos(Th6)*sin(Th2) - 0.0000414*cos(Th2)*cos(Th5)*sin(Th4)*sin(Th6) + 0.000013987*cos(Th2 + Th3)*cos(Th4)^2*cos(Th6)*sin(Th5) - 5.9869e-6*cos(Th2 + Th3)*cos(Th6)*sin(Th4)^2*sin(Th5) - 5.9735e-6*sin(Th2 + Th3)*cos(Th4)*cos(Th6)^2*sin(Th5) - 2.645e-8*sin(Th2 + Th3)*cos(Th4)*sin(Th5)*sin(Th6)^2 - 0.000013987*sin(Th2 + Th3)*cos(Th5)^2*sin(Th4)*sin(Th6) + 5.9869e-6*sin(Th2 + Th3)*sin(Th4)*sin(Th5)^2*sin(Th6) + 0.000011974*cos(Th2 + Th3)*cos(Th4)^2*cos(Th5)*cos(Th6)^2 + 2.645e-8*cos(Th2 + Th3)*cos(Th5)*cos(Th6)^2*sin(Th4)^2 + 2.645e-8*cos(Th2 + Th3)*cos(Th4)^2*cos(Th5)*sin(Th6)^2 - 2.645e-8*cos(Th2 + Th3)*cos(Th5)*sin(Th4)^2*sin(Th6)^2 - 0.00002921*cos(Th2)*cos(Th5)*sin(Th3)*sin(Th4)*sin(Th6) - 0.00002921*cos(Th3)*cos(Th5)*sin(Th2)*sin(Th4)*sin(Th6) - 5.9471e-6*cos(Th2 + Th3)*cos(Th4)*cos(Th6)*sin(Th4)*sin(Th6) - 0.000019974*cos(Th2 + Th3)*cos(Th4)*cos(Th5)*sin(Th4)*sin(Th5)*sin(Th6) + 5.9471e-6*sin(Th2 + Th3)*cos(Th5)*cos(Th6)*sin(Th4)*sin(Th5)*sin(Th6) - 5.9471e-6*cos(Th2 + Th3)*cos(Th4)*cos(Th5)^2*cos(Th6)*sin(Th4)*sin(Th6))*dTh2*dTh6;
%---------------------------
V131=(0)*dTh3*dTh1;
V132=V123;
V133=O123*dTh3*dTh3;
V134=(0.010223*cos(Th2 + Th3) - 1.0*(0.02603*cos(Th4)*sin(Th5) + 0.000115*sin(Th4)*sin(Th6) - 0.000115*cos(Th4)*cos(Th5)*cos(Th6))*(0.126*sin(Th2 + Th3) + 0.05206*sin(Th2 + Th3)*cos(Th5) + 0.254*cos(Th2)*sin(Th3) + 0.254*cos(Th3)*sin(Th2) + 0.05206*cos(Th2 + Th3)*cos(Th4)*sin(Th5) + 0.00023*cos(Th2 + Th3)*sin(Th4)*sin(Th6) + 0.00023*sin(Th2 + Th3)*cos(Th6)*sin(Th5) - 0.00023*cos(Th2 + Th3)*cos(Th4)*cos(Th5)*cos(Th6)) + 5.0e-11*cos(Th2 + Th3)*(23.0*cos(Th4)*sin(Th6) - 5206.0*sin(Th4)*sin(Th5) + 23.0*cos(Th5)*cos(Th6)*sin(Th4))^2 - 1.0*(0.00062*sin(Th4) + 0.00002*cos(Th4)*cos(Th5) - 0.00152*cos(Th4)*sin(Th5))*(0.126*sin(Th2 + Th3) + 0.00062*cos(Th2 + Th3)*sin(Th4) - 0.00152*sin(Th2 + Th3)*cos(Th5) - 0.00002*sin(Th2 + Th3)*sin(Th5) + 0.254*cos(Th2)*sin(Th3) + 0.254*cos(Th3)*sin(Th2) + 0.00002*cos(Th2 + Th3)*cos(Th4)*cos(Th5) - 0.00152*cos(Th2 + Th3)*cos(Th4)*sin(Th5)) - 0.020446*cos(Th2 + Th3)*cos(Th4)^2 - 0.005333*cos(Th2 + Th3)*cos(Th5)^2 - 3.0e-6*cos(Th2 + Th3)*cos(Th6)^2 + 4.0e-10*cos(Th2 + Th3)*(31.0*cos(Th4) - 1.0*cos(Th5)*sin(Th4) + 76.0*sin(Th4)*sin(Th5))^2 - 4.0e-6*sin(Th2 + Th3)*cos(Th4)*cos(Th6) - 0.00004*sin(Th2 + Th3)*cos(Th5)*sin(Th4) + 0.010666*cos(Th2 + Th3)*cos(Th4)^2*cos(Th5)^2 + 6.0e-6*cos(Th2 + Th3)*cos(Th4)^2*cos(Th6)^2 - 3.0e-6*cos(Th2 + Th3)*cos(Th5)^2*cos(Th6)^2 - 8.0e-6*cos(Th2 + Th3)*cos(Th5)*cos(Th6)*sin(Th5) + 6.0e-6*cos(Th2 + Th3)*cos(Th4)^2*cos(Th5)^2*cos(Th6)^2 - 0.00016*cos(Th2 + Th3)*cos(Th4)*sin(Th4)*sin(Th5) - 0.005333*sin(Th2 + Th3)*cos(Th4)*cos(Th5)*sin(Th5) - 4.0e-6*sin(Th2 + Th3)*cos(Th5)*sin(Th4)*sin(Th6) + 8.0e-6*sin(Th2 + Th3)*cos(Th4)*cos(Th5)^2*cos(Th6) + 0.000016*cos(Th2 + Th3)*cos(Th4)^2*cos(Th5)*cos(Th6)*sin(Th5) - 3.0e-6*sin(Th2 + Th3)*cos(Th4)*cos(Th5)*cos(Th6)^2*sin(Th5) - 0.000016*cos(Th2 + Th3)*cos(Th4)*sin(Th4)*sin(Th5)*sin(Th6) + 3.0e-6*sin(Th2 + Th3)*cos(Th6)*sin(Th4)*sin(Th5)*sin(Th6) - 0.000012*cos(Th2 + Th3)*cos(Th4)*cos(Th5)*cos(Th6)*sin(Th4)*sin(Th6))*dTh3*dTh4;
V135=(0.005333*sin(Th2 + Th3)*sin(Th4) - 0.00004*cos(Th2 + Th3)*cos(Th5) - 1.24e-8*sin(Th2 + Th3)*cos(Th4)*cos(Th5) - 4.0e-6*cos(Th2 + Th3)*cos(Th5)*sin(Th6) - 0.000039058*sin(Th2 + Th3)*cos(Th4)*sin(Th5) - 0.0030883*sin(Th2 + Th3)*cos(Th5)*sin(Th4) + 2.52e-6*sin(Th2 + Th3)*sin(Th4)*sin(Th5) + 0.000079058*cos(Th2 + Th3)*cos(Th4)^2*cos(Th5) + 9.424e-7*cos(Th2 + Th3)*cos(Th5)*sin(Th4)^2 - 1.24e-8*cos(Th2 + Th3)*cos(Th4)^2*sin(Th5) + 1.24e-8*cos(Th2 + Th3)*sin(Th4)^2*sin(Th5) - 0.012023*sin(Th2 + Th3)*cos(Th5)^2*sin(Th4) + 3.0e-6*sin(Th2 + Th3)*cos(Th6)^2*sin(Th4) + 0.0013574*sin(Th2 + Th3)*sin(Th4)*sin(Th5)^2 - 8.0e-6*cos(Th2 + Th3)*cos(Th4)*cos(Th6)*sin(Th4) + 3.0e-6*cos(Th2 + Th3)*cos(Th6)*sin(Th5)*sin(Th6) - 1.216e-7*sin(Th2 + Th3)*cos(Th5)*sin(Th4)*sin(Th5) - 9.9869e-6*sin(Th2 + Th3)*cos(Th4)*sin(Th5)*sin(Th6) - 0.00001449*sin(Th2 + Th3)*cos(Th6)*sin(Th4)*sin(Th5) - 0.0062255*cos(Th2)*cos(Th5)*sin(Th3)*sin(Th4) - 0.0062255*cos(Th3)*cos(Th5)*sin(Th2)*sin(Th4) + 6.08e-8*cos(Th2 + Th3)*cos(Th4)*cos(Th5)^2*sin(Th4) + 0.000013987*cos(Th2 + Th3)*cos(Th4)^2*cos(Th5)*sin(Th6) + 5.08e-6*cos(Th2)*sin(Th3)*sin(Th4)*sin(Th5) + 5.08e-6*cos(Th3)*sin(Th2)*sin(Th4)*sin(Th5) - 6.08e-8*cos(Th2 + Th3)*cos(Th4)*sin(Th4)*sin(Th5)^2 - 5.9869e-6*cos(Th2 + Th3)*cos(Th5)*sin(Th4)^2*sin(Th6) - 5.9735e-6*sin(Th2 + Th3)*cos(Th5)^2*cos(Th6)^2*sin(Th4) - 2.645e-8*sin(Th2 + Th3)*cos(Th6)^2*sin(Th4)*sin(Th5)^2 + 0.000027974*cos(Th2 + Th3)*cos(Th4)*cos(Th5)^2*cos(Th6)*sin(Th4) - 0.00002921*cos(Th2)*cos(Th6)*sin(Th3)*sin(Th4)*sin(Th5) - 0.00002921*cos(Th3)*cos(Th6)*sin(Th2)*sin(Th4)*sin(Th5) - 0.000011974*cos(Th2 + Th3)*cos(Th4)*cos(Th6)*sin(Th4)*sin(Th5)^2 - 5.9735e-6*cos(Th2 + Th3)*cos(Th4)^2*cos(Th6)*sin(Th5)*sin(Th6) - 2.645e-8*cos(Th2 + Th3)*cos(Th6)*sin(Th4)^2*sin(Th5)*sin(Th6) - 0.013381*cos(Th2 + Th3)*cos(Th4)*cos(Th5)*sin(Th4)*sin(Th5) - 2.9736e-6*sin(Th2 + Th3)*cos(Th4)*cos(Th5)*cos(Th6)*sin(Th6) - 0.000039948*sin(Th2 + Th3)*cos(Th5)*cos(Th6)*sin(Th4)*sin(Th5) - 5.9471e-6*cos(Th2 + Th3)*cos(Th4)*cos(Th5)*cos(Th6)^2*sin(Th4)*sin(Th5))*dTh3*dTh5;
V136=(3.0e-6*cos(Th2 + Th3)*cos(Th5) + 0.00001449*sin(Th2 + Th3)*cos(Th4)*cos(Th6) - 4.0e-6*cos(Th2 + Th3)*cos(Th6)*sin(Th5) + 3.0e-6*sin(Th2 + Th3)*cos(Th4)*sin(Th5) + 4.0e-6*sin(Th2 + Th3)*sin(Th4)*sin(Th6) - 6.0e-6*cos(Th2 + Th3)*cos(Th4)^2*cos(Th5) - 6.0e-6*cos(Th2 + Th3)*cos(Th5)*cos(Th6)^2 + 9.9869e-6*sin(Th2 + Th3)*cos(Th4)*cos(Th5)*cos(Th6) - 0.00001449*sin(Th2 + Th3)*cos(Th5)*sin(Th4)*sin(Th6) + 0.00002921*cos(Th2)*cos(Th4)*cos(Th6)*sin(Th3) + 0.00002921*cos(Th3)*cos(Th4)*cos(Th6)*sin(Th2) + 0.000013987*cos(Th2 + Th3)*cos(Th4)^2*cos(Th6)*sin(Th5) - 5.9869e-6*cos(Th2 + Th3)*cos(Th6)*sin(Th4)^2*sin(Th5) - 5.9735e-6*sin(Th2 + Th3)*cos(Th4)*cos(Th6)^2*sin(Th5) - 2.645e-8*sin(Th2 + Th3)*cos(Th4)*sin(Th5)*sin(Th6)^2 - 0.000013987*sin(Th2 + Th3)*cos(Th5)^2*sin(Th4)*sin(Th6) + 5.9869e-6*sin(Th2 + Th3)*sin(Th4)*sin(Th5)^2*sin(Th6) + 0.000011974*cos(Th2 + Th3)*cos(Th4)^2*cos(Th5)*cos(Th6)^2 + 2.645e-8*cos(Th2 + Th3)*cos(Th5)*cos(Th6)^2*sin(Th4)^2 + 2.645e-8*cos(Th2 + Th3)*cos(Th4)^2*cos(Th5)*sin(Th6)^2 - 2.645e-8*cos(Th2 + Th3)*cos(Th5)*sin(Th4)^2*sin(Th6)^2 - 0.00002921*cos(Th2)*cos(Th5)*sin(Th3)*sin(Th4)*sin(Th6) - 0.00002921*cos(Th3)*cos(Th5)*sin(Th2)*sin(Th4)*sin(Th6) - 5.9471e-6*cos(Th2 + Th3)*cos(Th4)*cos(Th6)*sin(Th4)*sin(Th6) - 0.000019974*cos(Th2 + Th3)*cos(Th4)*cos(Th5)*sin(Th4)*sin(Th5)*sin(Th6) + 5.9471e-6*sin(Th2 + Th3)*cos(Th5)*cos(Th6)*sin(Th4)*sin(Th5)*sin(Th6) - 5.9471e-6*cos(Th2 + Th3)*cos(Th4)*cos(Th5)^2*cos(Th6)*sin(Th4)*sin(Th6))*dTh3*dTh6;
%---------------------------
V141=(0)*dTh4*dTh1;
V142=(0.012239*cos(Th2)*cos(Th3) + 0.0002232*cos(Th2)*sin(Th4) - 0.012239*sin(Th2)*sin(Th3) + 0.0066904*cos(Th5)^2*sin(Th2)*sin(Th3) - 2.9736e-6*cos(Th6)^2*sin(Th2)*sin(Th3) + 7.2e-6*cos(Th2)*cos(Th4)*cos(Th5) + 3.04e-8*cos(Th2)*cos(Th4)*sin(Th3) + 3.04e-8*cos(Th3)*cos(Th4)*sin(Th2) + 0.0088236*cos(Th2)*cos(Th4)*sin(Th5) + 0.0002356*cos(Th2)*sin(Th3)*sin(Th4) + 0.0002356*cos(Th3)*sin(Th2)*sin(Th4) + 0.0000414*cos(Th2)*sin(Th4)*sin(Th6) - 0.0066904*cos(Th2)*cos(Th3)*cos(Th5)^2 + 2.9736e-6*cos(Th2)*cos(Th3)*cos(Th6)^2 + 2.9736e-6*cos(Th5)^2*cos(Th6)^2*sin(Th2)*sin(Th3) - 0.0000414*cos(Th2)*cos(Th4)*cos(Th5)*cos(Th6) + 7.6e-6*cos(Th2)*cos(Th4)*cos(Th5)*sin(Th3) + 7.6e-6*cos(Th3)*cos(Th4)*cos(Th5)*sin(Th2) - 6.08e-8*cos(Th2)*cos(Th3)*cos(Th5)*sin(Th5) + 9.9869e-6*cos(Th2)*cos(Th4)*cos(Th6)*sin(Th3) + 9.9869e-6*cos(Th3)*cos(Th4)*cos(Th6)*sin(Th2) + 0.0093138*cos(Th2)*cos(Th4)*sin(Th3)*sin(Th5) + 0.000039058*cos(Th2)*cos(Th5)*sin(Th3)*sin(Th4) + 0.0093138*cos(Th3)*cos(Th4)*sin(Th2)*sin(Th5) + 0.000039058*cos(Th3)*cos(Th5)*sin(Th2)*sin(Th4) - 1.24e-8*cos(Th2)*sin(Th3)*sin(Th4)*sin(Th5) - 1.24e-8*cos(Th3)*sin(Th2)*sin(Th4)*sin(Th5) + 0.0000437*cos(Th2)*sin(Th3)*sin(Th4)*sin(Th6) + 0.0000437*cos(Th3)*sin(Th2)*sin(Th4)*sin(Th6) + 6.08e-8*cos(Th5)*sin(Th2)*sin(Th3)*sin(Th5) - 6.08e-8*cos(Th2)*cos(Th4)*cos(Th5)^2*sin(Th3) - 6.08e-8*cos(Th3)*cos(Th4)*cos(Th5)^2*sin(Th2) - 2.9736e-6*cos(Th2)*cos(Th3)*cos(Th5)^2*cos(Th6)^2 - 0.0000437*cos(Th2)*cos(Th4)*cos(Th5)*cos(Th6)*sin(Th3) - 0.0000437*cos(Th3)*cos(Th4)*cos(Th5)*cos(Th6)*sin(Th2) - 0.000019974*cos(Th2)*cos(Th3)*cos(Th5)*cos(Th6)*sin(Th5) + 0.0066904*cos(Th2)*cos(Th4)*cos(Th5)*sin(Th3)*sin(Th5) + 0.0066904*cos(Th3)*cos(Th4)*cos(Th5)*sin(Th2)*sin(Th5) + 9.9869e-6*cos(Th2)*cos(Th5)*sin(Th3)*sin(Th4)*sin(Th6) + 9.9869e-6*cos(Th3)*cos(Th5)*sin(Th2)*sin(Th4)*sin(Th6) + 0.000019974*cos(Th5)*cos(Th6)*sin(Th2)*sin(Th3)*sin(Th5) - 0.000019974*cos(Th2)*cos(Th4)*cos(Th5)^2*cos(Th6)*sin(Th3) - 0.000019974*cos(Th3)*cos(Th4)*cos(Th5)^2*cos(Th6)*sin(Th2) + 2.9736e-6*cos(Th2)*cos(Th4)*cos(Th5)*cos(Th6)^2*sin(Th3)*sin(Th5) + 2.9736e-6*cos(Th3)*cos(Th4)*cos(Th5)*cos(Th6)^2*sin(Th2)*sin(Th5) - 2.9736e-6*cos(Th2)*cos(Th6)*sin(Th3)*sin(Th4)*sin(Th5)*sin(Th6) - 2.9736e-6*cos(Th3)*cos(Th6)*sin(Th2)*sin(Th4)*sin(Th5)*sin(Th6))*dTh4*dTh2;
V143=(0.012239*cos(Th2)*cos(Th3) - 0.012239*sin(Th2)*sin(Th3) + 0.0066904*cos(Th5)^2*sin(Th2)*sin(Th3) - 2.9736e-6*cos(Th6)^2*sin(Th2)*sin(Th3) + 3.04e-8*cos(Th2)*cos(Th4)*sin(Th3) + 3.04e-8*cos(Th3)*cos(Th4)*sin(Th2) + 0.0002356*cos(Th2)*sin(Th3)*sin(Th4) + 0.0002356*cos(Th3)*sin(Th2)*sin(Th4) - 0.0066904*cos(Th2)*cos(Th3)*cos(Th5)^2 + 2.9736e-6*cos(Th2)*cos(Th3)*cos(Th6)^2 + 2.9736e-6*cos(Th5)^2*cos(Th6)^2*sin(Th2)*sin(Th3) + 7.6e-6*cos(Th2)*cos(Th4)*cos(Th5)*sin(Th3) + 7.6e-6*cos(Th3)*cos(Th4)*cos(Th5)*sin(Th2) - 6.08e-8*cos(Th2)*cos(Th3)*cos(Th5)*sin(Th5) + 9.9869e-6*cos(Th2)*cos(Th4)*cos(Th6)*sin(Th3) + 9.9869e-6*cos(Th3)*cos(Th4)*cos(Th6)*sin(Th2) + 0.0093138*cos(Th2)*cos(Th4)*sin(Th3)*sin(Th5) + 0.000039058*cos(Th2)*cos(Th5)*sin(Th3)*sin(Th4) + 0.0093138*cos(Th3)*cos(Th4)*sin(Th2)*sin(Th5) + 0.000039058*cos(Th3)*cos(Th5)*sin(Th2)*sin(Th4) - 1.24e-8*cos(Th2)*sin(Th3)*sin(Th4)*sin(Th5) - 1.24e-8*cos(Th3)*sin(Th2)*sin(Th4)*sin(Th5) + 0.0000437*cos(Th2)*sin(Th3)*sin(Th4)*sin(Th6) + 0.0000437*cos(Th3)*sin(Th2)*sin(Th4)*sin(Th6) + 6.08e-8*cos(Th5)*sin(Th2)*sin(Th3)*sin(Th5) - 6.08e-8*cos(Th2)*cos(Th4)*cos(Th5)^2*sin(Th3) - 6.08e-8*cos(Th3)*cos(Th4)*cos(Th5)^2*sin(Th2) - 2.9736e-6*cos(Th2)*cos(Th3)*cos(Th5)^2*cos(Th6)^2 - 0.0000437*cos(Th2)*cos(Th4)*cos(Th5)*cos(Th6)*sin(Th3) - 0.0000437*cos(Th3)*cos(Th4)*cos(Th5)*cos(Th6)*sin(Th2) - 0.000019974*cos(Th2)*cos(Th3)*cos(Th5)*cos(Th6)*sin(Th5) + 0.0066904*cos(Th2)*cos(Th4)*cos(Th5)*sin(Th3)*sin(Th5) + 0.0066904*cos(Th3)*cos(Th4)*cos(Th5)*sin(Th2)*sin(Th5) + 9.9869e-6*cos(Th2)*cos(Th5)*sin(Th3)*sin(Th4)*sin(Th6) + 9.9869e-6*cos(Th3)*cos(Th5)*sin(Th2)*sin(Th4)*sin(Th6) + 0.000019974*cos(Th5)*cos(Th6)*sin(Th2)*sin(Th3)*sin(Th5) - 0.000019974*cos(Th2)*cos(Th4)*cos(Th5)^2*cos(Th6)*sin(Th3) - 0.000019974*cos(Th3)*cos(Th4)*cos(Th5)^2*cos(Th6)*sin(Th2) + 2.9736e-6*cos(Th2)*cos(Th4)*cos(Th5)*cos(Th6)^2*sin(Th3)*sin(Th5) + 2.9736e-6*cos(Th3)*cos(Th4)*cos(Th5)*cos(Th6)^2*sin(Th2)*sin(Th5) - 2.9736e-6*cos(Th2)*cos(Th6)*sin(Th3)*sin(Th4)*sin(Th5)*sin(Th6) - 2.9736e-6*cos(Th3)*cos(Th6)*sin(Th2)*sin(Th4)*sin(Th5)*sin(Th6))*dTh4*dTh3;
V144=(0.0002232*cos(Th4)*sin(Th2) - 0.0000434*cos(Th4) + 1.4e-6*cos(Th5)*sin(Th4) - 8.05e-6*cos(Th4)*sin(Th6) + 0.0017157*sin(Th4)*sin(Th5) - 0.0002356*cos(Th2)*cos(Th3)*cos(Th4) + 3.04e-8*cos(Th2)*cos(Th3)*sin(Th4) - 8.05e-6*cos(Th5)*cos(Th6)*sin(Th4) + 0.0002356*cos(Th4)*sin(Th2)*sin(Th3) - 7.2e-6*cos(Th5)*sin(Th2)*sin(Th4) + 0.0000414*cos(Th4)*sin(Th2)*sin(Th6) - 3.04e-8*sin(Th2)*sin(Th3)*sin(Th4) - 0.0088236*sin(Th2)*sin(Th4)*sin(Th5) - 0.000039058*cos(Th2)*cos(Th3)*cos(Th4)*cos(Th5) + 1.24e-8*cos(Th2)*cos(Th3)*cos(Th4)*sin(Th5) + 7.6e-6*cos(Th2)*cos(Th3)*cos(Th5)*sin(Th4) - 0.0000437*cos(Th2)*cos(Th3)*cos(Th4)*sin(Th6) + 9.9869e-6*cos(Th2)*cos(Th3)*cos(Th6)*sin(Th4) + 0.0093138*cos(Th2)*cos(Th3)*sin(Th4)*sin(Th5) + 0.000039058*cos(Th4)*cos(Th5)*sin(Th2)*sin(Th3) + 0.0000414*cos(Th5)*cos(Th6)*sin(Th2)*sin(Th4) - 1.24e-8*cos(Th4)*sin(Th2)*sin(Th3)*sin(Th5) - 7.6e-6*cos(Th5)*sin(Th2)*sin(Th3)*sin(Th4) + 0.0000437*cos(Th4)*sin(Th2)*sin(Th3)*sin(Th6) - 9.9869e-6*cos(Th6)*sin(Th2)*sin(Th3)*sin(Th4) - 0.0093138*sin(Th2)*sin(Th3)*sin(Th4)*sin(Th5) - 6.08e-8*cos(Th2)*cos(Th3)*cos(Th5)^2*sin(Th4) + 6.08e-8*cos(Th5)^2*sin(Th2)*sin(Th3)*sin(Th4) - 9.9869e-6*cos(Th2)*cos(Th3)*cos(Th4)*cos(Th5)*sin(Th6) - 0.0000437*cos(Th2)*cos(Th3)*cos(Th5)*cos(Th6)*sin(Th4) + 0.0066904*cos(Th2)*cos(Th3)*cos(Th5)*sin(Th4)*sin(Th5) + 9.9869e-6*cos(Th4)*cos(Th5)*sin(Th2)*sin(Th3)*sin(Th6) + 0.0000437*cos(Th5)*cos(Th6)*sin(Th2)*sin(Th3)*sin(Th4) - 0.0066904*cos(Th5)*sin(Th2)*sin(Th3)*sin(Th4)*sin(Th5) - 0.000019974*cos(Th2)*cos(Th3)*cos(Th5)^2*cos(Th6)*sin(Th4) + 0.000019974*cos(Th5)^2*cos(Th6)*sin(Th2)*sin(Th3)*sin(Th4) + 2.9736e-6*cos(Th2)*cos(Th3)*cos(Th5)*cos(Th6)^2*sin(Th4)*sin(Th5) - 2.9736e-6*cos(Th5)*cos(Th6)^2*sin(Th2)*sin(Th3)*sin(Th4)*sin(Th5) + 2.9736e-6*cos(Th2)*cos(Th3)*cos(Th4)*cos(Th6)*sin(Th5)*sin(Th6) - 2.9736e-6*cos(Th4)*cos(Th6)*sin(Th2)*sin(Th3)*sin(Th5)*sin(Th6))*dTh4*dTh4;
V145=(6.08e-8*cos(Th2)*sin(Th3) - 0.0017157*cos(Th4)*cos(Th5) + 6.08e-8*cos(Th3)*sin(Th2) + 1.4e-6*cos(Th4)*sin(Th5) + 0.0066904*cos(Th2)*cos(Th3)*cos(Th4) + 0.000019974*cos(Th2)*cos(Th6)*sin(Th3) + 0.000019974*cos(Th3)*cos(Th6)*sin(Th2) + 0.0088236*cos(Th4)*cos(Th5)*sin(Th2) - 8.05e-6*cos(Th4)*cos(Th6)*sin(Th5) - 0.0066904*cos(Th4)*sin(Th2)*sin(Th3) - 7.2e-6*cos(Th4)*sin(Th2)*sin(Th5) - 1.216e-7*cos(Th2)*cos(Th5)^2*sin(Th3) - 1.216e-7*cos(Th3)*cos(Th5)^2*sin(Th2) - 0.0093138*cos(Th2)*cos(Th3)*cos(Th4)*cos(Th5) + 7.6e-6*cos(Th2)*cos(Th3)*cos(Th4)*sin(Th5) + 1.24e-8*cos(Th2)*cos(Th3)*cos(Th5)*sin(Th4) + 0.000039058*cos(Th2)*cos(Th3)*sin(Th4)*sin(Th5) + 0.0093138*cos(Th4)*cos(Th5)*sin(Th2)*sin(Th3) + 0.013381*cos(Th2)*cos(Th5)*sin(Th3)*sin(Th5) + 0.013381*cos(Th3)*cos(Th5)*sin(Th2)*sin(Th5) + 0.0000414*cos(Th4)*cos(Th6)*sin(Th2)*sin(Th5) - 7.6e-6*cos(Th4)*sin(Th2)*sin(Th3)*sin(Th5) - 1.24e-8*cos(Th5)*sin(Th2)*sin(Th3)*sin(Th4) - 0.000039058*sin(Th2)*sin(Th3)*sin(Th4)*sin(Th5) - 0.013381*cos(Th2)*cos(Th3)*cos(Th4)*cos(Th5)^2 + 2.9736e-6*cos(Th2)*cos(Th3)*cos(Th4)*cos(Th6)^2 - 0.000039948*cos(Th2)*cos(Th5)^2*cos(Th6)*sin(Th3) - 0.000039948*cos(Th3)*cos(Th5)^2*cos(Th6)*sin(Th2) + 0.013381*cos(Th4)*cos(Th5)^2*sin(Th2)*sin(Th3) - 2.9736e-6*cos(Th4)*cos(Th6)^2*sin(Th2)*sin(Th3) - 1.216e-7*cos(Th2)*cos(Th3)*cos(Th4)*cos(Th5)*sin(Th5) - 0.0000437*cos(Th2)*cos(Th3)*cos(Th4)*cos(Th6)*sin(Th5) + 1.216e-7*cos(Th4)*cos(Th5)*sin(Th2)*sin(Th3)*sin(Th5) + 9.9869e-6*cos(Th2)*cos(Th3)*sin(Th4)*sin(Th5)*sin(Th6) + 0.0000437*cos(Th4)*cos(Th6)*sin(Th2)*sin(Th3)*sin(Th5) - 9.9869e-6*sin(Th2)*sin(Th3)*sin(Th4)*sin(Th5)*sin(Th6) + 5.9471e-6*cos(Th2)*cos(Th5)*cos(Th6)^2*sin(Th3)*sin(Th5) + 5.9471e-6*cos(Th3)*cos(Th5)*cos(Th6)^2*sin(Th2)*sin(Th5) - 5.9471e-6*cos(Th2)*cos(Th3)*cos(Th4)*cos(Th5)^2*cos(Th6)^2 + 5.9471e-6*cos(Th4)*cos(Th5)^2*cos(Th6)^2*sin(Th2)*sin(Th3) - 0.000039948*cos(Th2)*cos(Th3)*cos(Th4)*cos(Th5)*cos(Th6)*sin(Th5) + 2.9736e-6*cos(Th2)*cos(Th3)*cos(Th5)*cos(Th6)*sin(Th4)*sin(Th6) + 0.000039948*cos(Th4)*cos(Th5)*cos(Th6)*sin(Th2)*sin(Th3)*sin(Th5) - 2.9736e-6*cos(Th5)*cos(Th6)*sin(Th2)*sin(Th3)*sin(Th4)*sin(Th6))*dTh4*dTh5;
V146=(0.0000414*cos(Th6)*sin(Th2)*sin(Th4) - 8.05e-6*cos(Th4)*cos(Th5)*sin(Th6) - 8.05e-6*cos(Th6)*sin(Th4) + 9.9869e-6*cos(Th2)*cos(Th3)*cos(Th4)*sin(Th6) - 0.0000437*cos(Th2)*cos(Th3)*cos(Th6)*sin(Th4) - 2.9736e-6*cos(Th2)*cos(Th3)*sin(Th4)*sin(Th5) - 5.9471e-6*cos(Th2)*cos(Th6)*sin(Th3)*sin(Th6) - 5.9471e-6*cos(Th3)*cos(Th6)*sin(Th2)*sin(Th6) + 0.0000414*cos(Th4)*cos(Th5)*sin(Th2)*sin(Th6) - 9.9869e-6*cos(Th4)*sin(Th2)*sin(Th3)*sin(Th6) + 0.0000437*cos(Th6)*sin(Th2)*sin(Th3)*sin(Th4) + 2.9736e-6*sin(Th2)*sin(Th3)*sin(Th4)*sin(Th5) - 0.0000437*cos(Th2)*cos(Th3)*cos(Th4)*cos(Th5)*sin(Th6) - 9.9869e-6*cos(Th2)*cos(Th3)*cos(Th5)*cos(Th6)*sin(Th4) + 0.0000437*cos(Th4)*cos(Th5)*sin(Th2)*sin(Th3)*sin(Th6) + 9.9869e-6*cos(Th5)*cos(Th6)*sin(Th2)*sin(Th3)*sin(Th4) + 0.000019974*cos(Th2)*cos(Th5)*sin(Th3)*sin(Th5)*sin(Th6) + 0.000019974*cos(Th3)*cos(Th5)*sin(Th2)*sin(Th5)*sin(Th6) - 0.000019974*cos(Th2)*cos(Th3)*cos(Th4)*cos(Th5)^2*sin(Th6) + 5.9471e-6*cos(Th2)*cos(Th3)*cos(Th6)^2*sin(Th4)*sin(Th5) + 5.9471e-6*cos(Th2)*cos(Th5)^2*cos(Th6)*sin(Th3)*sin(Th6) + 5.9471e-6*cos(Th3)*cos(Th5)^2*cos(Th6)*sin(Th2)*sin(Th6) + 0.000019974*cos(Th4)*cos(Th5)^2*sin(Th2)*sin(Th3)*sin(Th6) - 5.9471e-6*cos(Th6)^2*sin(Th2)*sin(Th3)*sin(Th4)*sin(Th5) + 5.9471e-6*cos(Th2)*cos(Th3)*cos(Th4)*cos(Th5)*cos(Th6)*sin(Th5)*sin(Th6) - 5.9471e-6*cos(Th4)*cos(Th5)*cos(Th6)*sin(Th2)*sin(Th3)*sin(Th5)*sin(Th6))*dTh4*dTh6;
%---------------------------
V151=(0)*dTh5*dTh1;
V152=(0.000039058*cos(Th2)*cos(Th3)*cos(Th5) - 1.24e-8*cos(Th2)*cos(Th3)*sin(Th5) + 0.0088236*cos(Th2)*cos(Th5)*sin(Th4) + 0.0075924*cos(Th2)*sin(Th3)*sin(Th4) + 0.0075924*cos(Th3)*sin(Th2)*sin(Th4) - 0.000039058*cos(Th5)*sin(Th2)*sin(Th3) - 7.2e-6*cos(Th2)*sin(Th4)*sin(Th5) + 1.24e-8*sin(Th2)*sin(Th3)*sin(Th5) - 1.24e-8*cos(Th2)*cos(Th4)*cos(Th5)*sin(Th3) - 1.24e-8*cos(Th3)*cos(Th4)*cos(Th5)*sin(Th2) + 9.9869e-6*cos(Th2)*cos(Th3)*cos(Th5)*sin(Th6) - 0.000039058*cos(Th2)*cos(Th4)*sin(Th3)*sin(Th5) + 0.0093138*cos(Th2)*cos(Th5)*sin(Th3)*sin(Th4) - 0.000039058*cos(Th3)*cos(Th4)*sin(Th2)*sin(Th5) + 0.0093138*cos(Th3)*cos(Th5)*sin(Th2)*sin(Th4) + 0.0000414*cos(Th2)*cos(Th6)*sin(Th4)*sin(Th5) - 7.6e-6*cos(Th2)*sin(Th3)*sin(Th4)*sin(Th5) - 7.6e-6*cos(Th3)*sin(Th2)*sin(Th4)*sin(Th5) - 9.9869e-6*cos(Th5)*sin(Th2)*sin(Th3)*sin(Th6) - 2.9736e-6*cos(Th2)*cos(Th6)^2*sin(Th3)*sin(Th4) - 2.9736e-6*cos(Th3)*cos(Th6)^2*sin(Th2)*sin(Th4) - 2.9736e-6*cos(Th2)*cos(Th3)*cos(Th6)*sin(Th5)*sin(Th6) - 9.9869e-6*cos(Th2)*cos(Th4)*sin(Th3)*sin(Th5)*sin(Th6) + 0.0000437*cos(Th2)*cos(Th6)*sin(Th3)*sin(Th4)*sin(Th5) - 9.9869e-6*cos(Th3)*cos(Th4)*sin(Th2)*sin(Th5)*sin(Th6) + 0.0000437*cos(Th3)*cos(Th6)*sin(Th2)*sin(Th4)*sin(Th5) + 2.9736e-6*cos(Th6)*sin(Th2)*sin(Th3)*sin(Th5)*sin(Th6) - 2.9736e-6*cos(Th2)*cos(Th4)*cos(Th5)*cos(Th6)*sin(Th3)*sin(Th6) - 2.9736e-6*cos(Th3)*cos(Th4)*cos(Th5)*cos(Th6)*sin(Th2)*sin(Th6))*dTh5*dTh2;
V153=(0.000039058*cos(Th2)*cos(Th3)*cos(Th5) - 1.24e-8*cos(Th2)*cos(Th3)*sin(Th5) + 0.0075924*cos(Th2)*sin(Th3)*sin(Th4) + 0.0075924*cos(Th3)*sin(Th2)*sin(Th4) - 0.000039058*cos(Th5)*sin(Th2)*sin(Th3) + 1.24e-8*sin(Th2)*sin(Th3)*sin(Th5) - 1.24e-8*cos(Th2)*cos(Th4)*cos(Th5)*sin(Th3) - 1.24e-8*cos(Th3)*cos(Th4)*cos(Th5)*sin(Th2) + 9.9869e-6*cos(Th2)*cos(Th3)*cos(Th5)*sin(Th6) - 0.000039058*cos(Th2)*cos(Th4)*sin(Th3)*sin(Th5) + 0.0093138*cos(Th2)*cos(Th5)*sin(Th3)*sin(Th4) - 0.000039058*cos(Th3)*cos(Th4)*sin(Th2)*sin(Th5) + 0.0093138*cos(Th3)*cos(Th5)*sin(Th2)*sin(Th4) - 7.6e-6*cos(Th2)*sin(Th3)*sin(Th4)*sin(Th5) - 7.6e-6*cos(Th3)*sin(Th2)*sin(Th4)*sin(Th5) - 9.9869e-6*cos(Th5)*sin(Th2)*sin(Th3)*sin(Th6) - 2.9736e-6*cos(Th2)*cos(Th6)^2*sin(Th3)*sin(Th4) - 2.9736e-6*cos(Th3)*cos(Th6)^2*sin(Th2)*sin(Th4) - 2.9736e-6*cos(Th2)*cos(Th3)*cos(Th6)*sin(Th5)*sin(Th6) - 9.9869e-6*cos(Th2)*cos(Th4)*sin(Th3)*sin(Th5)*sin(Th6) + 0.0000437*cos(Th2)*cos(Th6)*sin(Th3)*sin(Th4)*sin(Th5) - 9.9869e-6*cos(Th3)*cos(Th4)*sin(Th2)*sin(Th5)*sin(Th6) + 0.0000437*cos(Th3)*cos(Th6)*sin(Th2)*sin(Th4)*sin(Th5) + 2.9736e-6*cos(Th6)*sin(Th2)*sin(Th3)*sin(Th5)*sin(Th6) - 2.9736e-6*cos(Th2)*cos(Th4)*cos(Th5)*cos(Th6)*sin(Th3)*sin(Th6) - 2.9736e-6*cos(Th3)*cos(Th4)*cos(Th5)*cos(Th6)*sin(Th2)*sin(Th6))*dTh5*dTh3;
V154=(1.4e-6*cos(Th4)*sin(Th5) - 0.0017157*cos(Th4)*cos(Th5) - 0.0075924*cos(Th2)*cos(Th3)*cos(Th4) + 0.0088236*cos(Th4)*cos(Th5)*sin(Th2) - 8.05e-6*cos(Th4)*cos(Th6)*sin(Th5) + 0.0075924*cos(Th4)*sin(Th2)*sin(Th3) - 7.2e-6*cos(Th4)*sin(Th2)*sin(Th5) - 0.0093138*cos(Th2)*cos(Th3)*cos(Th4)*cos(Th5) + 7.6e-6*cos(Th2)*cos(Th3)*cos(Th4)*sin(Th5) - 1.24e-8*cos(Th2)*cos(Th3)*cos(Th5)*sin(Th4) - 0.000039058*cos(Th2)*cos(Th3)*sin(Th4)*sin(Th5) + 0.0093138*cos(Th4)*cos(Th5)*sin(Th2)*sin(Th3) + 0.0000414*cos(Th4)*cos(Th6)*sin(Th2)*sin(Th5) - 7.6e-6*cos(Th4)*sin(Th2)*sin(Th3)*sin(Th5) + 1.24e-8*cos(Th5)*sin(Th2)*sin(Th3)*sin(Th4) + 0.000039058*sin(Th2)*sin(Th3)*sin(Th4)*sin(Th5) + 2.9736e-6*cos(Th2)*cos(Th3)*cos(Th4)*cos(Th6)^2 - 2.9736e-6*cos(Th4)*cos(Th6)^2*sin(Th2)*sin(Th3) - 0.0000437*cos(Th2)*cos(Th3)*cos(Th4)*cos(Th6)*sin(Th5) - 9.9869e-6*cos(Th2)*cos(Th3)*sin(Th4)*sin(Th5)*sin(Th6) + 0.0000437*cos(Th4)*cos(Th6)*sin(Th2)*sin(Th3)*sin(Th5) + 9.9869e-6*sin(Th2)*sin(Th3)*sin(Th4)*sin(Th5)*sin(Th6) - 2.9736e-6*cos(Th2)*cos(Th3)*cos(Th5)*cos(Th6)*sin(Th4)*sin(Th6) + 2.9736e-6*cos(Th5)*cos(Th6)*sin(Th2)*sin(Th3)*sin(Th4)*sin(Th6))*dTh5*dTh4;
V155=(1.4e-6*cos(Th5)*sin(Th4) + 0.0017157*sin(Th4)*sin(Th5) - 1.24e-8*cos(Th2)*cos(Th5)*sin(Th3) - 1.24e-8*cos(Th3)*cos(Th5)*sin(Th2) - 8.05e-6*cos(Th5)*cos(Th6)*sin(Th4) - 0.000039058*cos(Th2)*sin(Th3)*sin(Th5) - 0.000039058*cos(Th3)*sin(Th2)*sin(Th5) - 7.2e-6*cos(Th5)*sin(Th2)*sin(Th4) - 0.0088236*sin(Th2)*sin(Th4)*sin(Th5) + 0.000039058*cos(Th2)*cos(Th3)*cos(Th4)*cos(Th5) - 1.24e-8*cos(Th2)*cos(Th3)*cos(Th4)*sin(Th5) + 7.6e-6*cos(Th2)*cos(Th3)*cos(Th5)*sin(Th4) + 0.0093138*cos(Th2)*cos(Th3)*sin(Th4)*sin(Th5) - 0.000039058*cos(Th4)*cos(Th5)*sin(Th2)*sin(Th3) + 0.0000414*cos(Th5)*cos(Th6)*sin(Th2)*sin(Th4) + 1.24e-8*cos(Th4)*sin(Th2)*sin(Th3)*sin(Th5) - 7.6e-6*cos(Th5)*sin(Th2)*sin(Th3)*sin(Th4) - 9.9869e-6*cos(Th2)*sin(Th3)*sin(Th5)*sin(Th6) - 9.9869e-6*cos(Th3)*sin(Th2)*sin(Th5)*sin(Th6) - 0.0093138*sin(Th2)*sin(Th3)*sin(Th4)*sin(Th5) + 9.9869e-6*cos(Th2)*cos(Th3)*cos(Th4)*cos(Th5)*sin(Th6) - 0.0000437*cos(Th2)*cos(Th3)*cos(Th5)*cos(Th6)*sin(Th4) - 2.9736e-6*cos(Th2)*cos(Th5)*cos(Th6)*sin(Th3)*sin(Th6) - 2.9736e-6*cos(Th3)*cos(Th5)*cos(Th6)*sin(Th2)*sin(Th6) - 9.9869e-6*cos(Th4)*cos(Th5)*sin(Th2)*sin(Th3)*sin(Th6) + 0.0000437*cos(Th5)*cos(Th6)*sin(Th2)*sin(Th3)*sin(Th4) - 2.9736e-6*cos(Th2)*cos(Th3)*cos(Th4)*cos(Th6)*sin(Th5)*sin(Th6) + 2.9736e-6*cos(Th4)*cos(Th6)*sin(Th2)*sin(Th3)*sin(Th5)*sin(Th6))*dTh5*dTh5;
V156=(2.9736e-6*cos(Th2)*sin(Th3)*sin(Th5) + 2.9736e-6*cos(Th3)*sin(Th2)*sin(Th5) + 8.05e-6*sin(Th4)*sin(Th5)*sin(Th6) - 2.9736e-6*cos(Th2)*cos(Th3)*cos(Th4)*cos(Th5) + 9.9869e-6*cos(Th2)*cos(Th5)*cos(Th6)*sin(Th3) + 9.9869e-6*cos(Th3)*cos(Th5)*cos(Th6)*sin(Th2) + 2.9736e-6*cos(Th4)*cos(Th5)*sin(Th2)*sin(Th3) - 0.0000414*sin(Th2)*sin(Th4)*sin(Th5)*sin(Th6) - 5.9471e-6*cos(Th2)*cos(Th6)^2*sin(Th3)*sin(Th5) - 5.9471e-6*cos(Th3)*cos(Th6)^2*sin(Th2)*sin(Th5) + 9.9869e-6*cos(Th2)*cos(Th3)*cos(Th4)*cos(Th6)*sin(Th5) - 5.9471e-6*cos(Th2)*cos(Th3)*cos(Th6)*sin(Th4)*sin(Th6) + 0.0000437*cos(Th2)*cos(Th3)*sin(Th4)*sin(Th5)*sin(Th6) - 9.9869e-6*cos(Th4)*cos(Th6)*sin(Th2)*sin(Th3)*sin(Th5) + 5.9471e-6*cos(Th6)*sin(Th2)*sin(Th3)*sin(Th4)*sin(Th6) - 0.0000437*sin(Th2)*sin(Th3)*sin(Th4)*sin(Th5)*sin(Th6) + 5.9471e-6*cos(Th2)*cos(Th3)*cos(Th4)*cos(Th5)*cos(Th6)^2 - 5.9471e-6*cos(Th4)*cos(Th5)*cos(Th6)^2*sin(Th2)*sin(Th3))*dTh5*dTh6;
%---------------------------
V161=(0)*dTh6*dTh1;
V162=(0.00011603*cos(Th2)*cos(Th3)*cos(Th5) - 0.0000414*cos(Th2)*cos(Th4)*cos(Th6) - 0.00011603*cos(Th5)*sin(Th2)*sin(Th3) - 0.0000437*cos(Th2)*cos(Th4)*cos(Th6)*sin(Th3) - 0.0000437*cos(Th3)*cos(Th4)*cos(Th6)*sin(Th2) - 9.9869e-6*cos(Th2)*cos(Th3)*cos(Th6)*sin(Th5) - 0.00011603*cos(Th2)*cos(Th4)*sin(Th3)*sin(Th5) - 0.00011603*cos(Th3)*cos(Th4)*sin(Th2)*sin(Th5) + 0.0000414*cos(Th2)*cos(Th5)*sin(Th4)*sin(Th6) + 9.9869e-6*cos(Th2)*sin(Th3)*sin(Th4)*sin(Th6) + 9.9869e-6*cos(Th3)*sin(Th2)*sin(Th4)*sin(Th6) + 9.9869e-6*cos(Th6)*sin(Th2)*sin(Th3)*sin(Th5) - 9.9869e-6*cos(Th2)*cos(Th4)*cos(Th5)*cos(Th6)*sin(Th3) - 9.9869e-6*cos(Th3)*cos(Th4)*cos(Th5)*cos(Th6)*sin(Th2) + 0.0000437*cos(Th2)*cos(Th5)*sin(Th3)*sin(Th4)*sin(Th6) + 0.0000437*cos(Th3)*cos(Th5)*sin(Th2)*sin(Th4)*sin(Th6))*dTh6*dTh2;
V163=(0.00011603*cos(Th2)*cos(Th3)*cos(Th5) - 0.00011603*cos(Th5)*sin(Th2)*sin(Th3) - 0.0000437*cos(Th2)*cos(Th4)*cos(Th6)*sin(Th3) - 0.0000437*cos(Th3)*cos(Th4)*cos(Th6)*sin(Th2) - 9.9869e-6*cos(Th2)*cos(Th3)*cos(Th6)*sin(Th5) - 0.00011603*cos(Th2)*cos(Th4)*sin(Th3)*sin(Th5) - 0.00011603*cos(Th3)*cos(Th4)*sin(Th2)*sin(Th5) + 9.9869e-6*cos(Th2)*sin(Th3)*sin(Th4)*sin(Th6) + 9.9869e-6*cos(Th3)*sin(Th2)*sin(Th4)*sin(Th6) + 9.9869e-6*cos(Th6)*sin(Th2)*sin(Th3)*sin(Th5) - 9.9869e-6*cos(Th2)*cos(Th4)*cos(Th5)*cos(Th6)*sin(Th3) - 9.9869e-6*cos(Th3)*cos(Th4)*cos(Th5)*cos(Th6)*sin(Th2) + 0.0000437*cos(Th2)*cos(Th5)*sin(Th3)*sin(Th4)*sin(Th6) + 0.0000437*cos(Th3)*cos(Th5)*sin(Th2)*sin(Th4)*sin(Th6))*dTh6*dTh3;
V164=(0.0000414*cos(Th6)*sin(Th2)*sin(Th4) - 8.05e-6*cos(Th4)*cos(Th5)*sin(Th6) - 8.05e-6*cos(Th6)*sin(Th4) - 9.9869e-6*cos(Th2)*cos(Th3)*cos(Th4)*sin(Th6) - 0.0000437*cos(Th2)*cos(Th3)*cos(Th6)*sin(Th4) - 0.00011603*cos(Th2)*cos(Th3)*sin(Th4)*sin(Th5) + 0.0000414*cos(Th4)*cos(Th5)*sin(Th2)*sin(Th6) + 9.9869e-6*cos(Th4)*sin(Th2)*sin(Th3)*sin(Th6) + 0.0000437*cos(Th6)*sin(Th2)*sin(Th3)*sin(Th4) + 0.00011603*sin(Th2)*sin(Th3)*sin(Th4)*sin(Th5) - 0.0000437*cos(Th2)*cos(Th3)*cos(Th4)*cos(Th5)*sin(Th6) - 9.9869e-6*cos(Th2)*cos(Th3)*cos(Th5)*cos(Th6)*sin(Th4) + 0.0000437*cos(Th4)*cos(Th5)*sin(Th2)*sin(Th3)*sin(Th6) + 9.9869e-6*cos(Th5)*cos(Th6)*sin(Th2)*sin(Th3)*sin(Th4))*dTh6*dTh4;
V165=(8.05e-6*sin(Th4)*sin(Th5)*sin(Th6) - 0.00011603*cos(Th3)*sin(Th2)*sin(Th5) - 0.00011603*cos(Th2)*sin(Th3)*sin(Th5) + 0.00011603*cos(Th2)*cos(Th3)*cos(Th4)*cos(Th5) - 9.9869e-6*cos(Th2)*cos(Th5)*cos(Th6)*sin(Th3) - 9.9869e-6*cos(Th3)*cos(Th5)*cos(Th6)*sin(Th2) - 0.00011603*cos(Th4)*cos(Th5)*sin(Th2)*sin(Th3) - 0.0000414*sin(Th2)*sin(Th4)*sin(Th5)*sin(Th6) - 9.9869e-6*cos(Th2)*cos(Th3)*cos(Th4)*cos(Th6)*sin(Th5) + 0.0000437*cos(Th2)*cos(Th3)*sin(Th4)*sin(Th5)*sin(Th6) + 9.9869e-6*cos(Th4)*cos(Th6)*sin(Th2)*sin(Th3)*sin(Th5) - 0.0000437*sin(Th2)*sin(Th3)*sin(Th4)*sin(Th5)*sin(Th6))*dTh6*dTh5;
V166=(0.0000414*cos(Th4)*sin(Th2)*sin(Th6) - 8.05e-6*cos(Th5)*cos(Th6)*sin(Th4) - 8.05e-6*cos(Th4)*sin(Th6) - 0.0000437*cos(Th2)*cos(Th3)*cos(Th4)*sin(Th6) - 9.9869e-6*cos(Th2)*cos(Th3)*cos(Th6)*sin(Th4) + 0.0000414*cos(Th5)*cos(Th6)*sin(Th2)*sin(Th4) + 0.0000437*cos(Th4)*sin(Th2)*sin(Th3)*sin(Th6) + 9.9869e-6*cos(Th6)*sin(Th2)*sin(Th3)*sin(Th4) + 9.9869e-6*cos(Th2)*sin(Th3)*sin(Th5)*sin(Th6) + 9.9869e-6*cos(Th3)*sin(Th2)*sin(Th5)*sin(Th6) - 9.9869e-6*cos(Th2)*cos(Th3)*cos(Th4)*cos(Th5)*sin(Th6) - 0.0000437*cos(Th2)*cos(Th3)*cos(Th5)*cos(Th6)*sin(Th4) + 9.9869e-6*cos(Th4)*cos(Th5)*sin(Th2)*sin(Th3)*sin(Th6) + 0.0000437*cos(Th5)*cos(Th6)*sin(Th2)*sin(Th3)*sin(Th4))*dTh6*dTh6;
%---------------------------
V1 = V111+V112+V113+V114+V115+V116+V121+V122+V123+V124+V125+V126+...
     V131+V132+V133+V134+V135+V136+V141+V142+V143+V144+V145+V146+...
     V151+V152+V153+V154+V155+V156+V161+V162+V163+V164+V165+V166;
end
